simulink model "lss"  (R2022b)
settings: Solver=FixedStepAuto  StartTime=0.0  StopTime=Inf  FixedStep=0.001  RelTol=1e-3  EnableMultiTasking=on
InitFcn:
  | clear mex
model workspace (MAT data in the model file):
  worldsim_instance : object (value not decoded)
values from neighbouring files (symbols this model uses):
  ADAS_Control_Mode = 1    [LSS_parameters.m]    (also in lss_ini_param.sldd = 1.0)
  butter_a = 1.0 -1.9911142922016536 0.99115359586893548    [lss_ini_param.sldd]
  butter_a_lka_out = 1.0 -1.5610180758007179 0.641351538057563    [lss_ini_param.sldd]
  butter_b = 9.825916820482009E-6 1.9651833640964018E-5 9.825916820482009E-6    [lss_ini_param.sldd]
  butter_b_lka_out = 0.020083365564211246 0.040166731128422492 0.020083365564211246    [lss_ini_param.sldd]
  index_variant_approaching_speed = 3.0    [lss_ini_param.sldd]
  initCond = vi_worldsim_load_scenario(worldsim_process,scenario_path,'lss_online')    [launcher.m]
  LDW_Activity_Flag = 1    [LSS_parameters.m]    (also in lss_ini_param.sldd = 1.0)
  LDW_Freq_Hz = Sensor_Freq_worldsim    [LSS_parameters.m]    (also in lss_ini_param.sldd = 50.0)
  LDW_LaneGap_dydt_Warning = 50    [LSS_parameters.m]    (also in lss_ini_param.sldd = 50.0)
  LDW_LaneGap_Warning = [0.5 0.25]    [LSS_parameters.m]    (also in lss_ini_param.sldd = 0.5 0.25)
  LDW_Min_Speed = 60    [LSS_parameters.m]    (also in lss_ini_param.sldd = 60.0)
  LDW_Steer_Vibration_Amplitude = 5    [LSS_parameters.m]    (also in lss_ini_param.sldd = 5.0)
  LDW_Steer_Vibration_Freq = 25    [LSS_parameters.m]    (also in lss_ini_param.sldd = 25.0)
  LKA_Activity_Flag = 1    [LSS_parameters.m]    (also in lss_ini_param.sldd = 1.0)
  LKA_D = [0.2 0.3]    [LSS_parameters.m]    (also in lss_ini_param.sldd = 0.2 0.3)
  LKA_Dyn_Rate_Limiter_Gain = 0.1    [LSS_parameters.m]    (also in lss_ini_param.sldd)
  LKA_Dyn_Rate_Limiter_Power = 10    [LSS_parameters.m]    (also in lss_ini_param.sldd = 10.0)
  LKA_Error_dydt_Off = 1    [LSS_parameters.m]    (also in lss_ini_param.sldd = 1.0)
  LKA_Error_Max = 3    [LSS_parameters.m]    (also in lss_ini_param.sldd = 3.0)
  LKA_Error_Off = 0.5    [LSS_parameters.m]    (also in lss_ini_param.sldd)
  LKA_Freq_Hz = Sensor_Freq_worldsim    [LSS_parameters.m]    (also in lss_ini_param.sldd = 50.0)
  LKA_I = [0.025 0.05]    [LSS_parameters.m]    (also in lss_ini_param.sldd = 0.025 0.05)
  LKA_Lane_Gap_Activate = [0.25 0.125]    [LSS_parameters.m]    (also in lss_ini_param.sldd = -0.05 0.125)
  LKA_Lane_Gap_dydt_Activate = 50    [LSS_parameters.m]    (also in lss_ini_param.sldd = 50.0)
  LKA_Min_Speed = 60    [LSS_parameters.m]    (also in lss_ini_param.mat = 50; lss_ini_param.sldd = 50.0)
  LKA_On_Display_Freq = 5    [LSS_parameters.m]    (also in lss_ini_param.sldd = 5.0)
  LKA_P = [0.1 0.2]    [LSS_parameters.m]    (also in lss_ini_param.sldd = 0.1 0.2)
  LKA_Steer_Rate_Max_radps = 1    [LSS_parameters.m]    (also in lss_ini_param.sldd = 1.0)
  radar_source = 2    [LSS_parameters.m]    (also in lss_ini_param.sldd = 2.0)
  Sensor_Freq_worldsim = 50    [launcher.m]    (also in lss_ini_param.sldd = 50.0)
  simulation_crt = '../VI-CarRealTime_model/SedanCar_WorldSim_Offline_send_svm.xml'    [launcher.m]
  stop_number_collisions = 5    [launcher.m]
  stop_speed = 0.001    [launcher.m]
  stop_time = 20    [launcher.m]
  target_speed = 72    [LSS_parameters.m]    (also in launcher.m = initCond.initialVelocity * 3.6)
  variant_approaching_speed = v_lat    [launcher.m]    (also in lss_ini_param.sldd = 0.2 0.3 0.4 0.5 0.6)
  vehicle_width = 1.86    [LSS_parameters.m]    (also in lss_ini_param.sldd = 2.05)
undefined symbols (not defined in the file or in its folder): Driver_Demands, light_brake_center, light_brake_left, light_brake_right, steer_assist, vicrt_initcallback, vicrt_initmexcallback, vicrt_simulationmanager
libraries: simulink x39, simwbSfunlib x15, viworldsim_lib x5
(part 3 of 6)

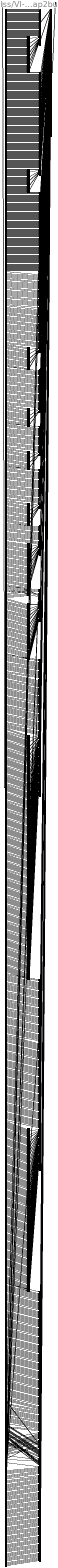
== system lss/VI-CarRealTime/Output_Bus/IOmap2bus ==
  In : Inport
  ABS_Activity : BusCreator  Inputs=4
  Actual_Tread_Speed : BusCreator  Inputs=4
  Aggregate_Force_At_Wheel : BusCreator  Inputs=4
  Alpha : BusCreator  Inputs=4
  Animator_Widget : BusCreator  Inputs=2
  Auxiliary_Roll_Force : BusCreator  Inputs=4
  Auxiliary_Roll_Force_at_element : BusCreator  Inputs=2
  Auxiliary_Roll_deformation_at_element : BusCreator  Inputs=2
  Brake : BusCreator  Inputs=8
  Brake_Moment : BusCreator  Inputs=4
  Caster_Angle : BusCreator  Inputs=2
  Chamber_Pressure : BusCreator  Inputs=4
  Contact_Flag : BusCreator  Inputs=4
  Contact_Patch_Global_X : BusCreator  Inputs=4
  Contact_Patch_Global_X1 : BusCreator  Inputs=4
  Contact_Patch_Global_Y : BusCreator  Inputs=4
  Contact_Patch_Global_Y1 : BusCreator  Inputs=4
  Contact_Patch_Global_Z : BusCreator  Inputs=4
  Contact_Patch_Global_Z1 : BusCreator  Inputs=4
  Contact_Patch_Normal_X : BusCreator  Inputs=4
  Contact_Patch_Normal_Y : BusCreator  Inputs=4
  Contact_Patch_Normal_Z : BusCreator  Inputs=4
  Damper : BusCreator  Inputs=5
  Demux : Demux  Outputs=1377
  Drive_Moment : BusCreator  Inputs=4
  Effective_Closing_Speed : BusCreator  Inputs=4
  Effective_Penetration : BusCreator  Inputs=4
  Effective_Rolling_Radius : BusCreator  Inputs=4
  Equivalent_Tread_Speed : BusCreator  Inputs=4
  Euler_Roll : BusCreator  Inputs=4
  External_Friction_Scale_Factor : BusCreator  Inputs=4
  Force_At_Bumper : BusCreator  Inputs=4
  Force_At_Bumper1 : BusCreator  Inputs=4
  Force_At_Damper : BusCreator  Inputs=4
  Force_At_Inerter : BusCreator  Inputs=4
  Force_At_Spring : BusCreator  Inputs=4
  Force_At_Wheel{,1..4} (5 alike) : BusCreator  Inputs=4
  Force_Aux_At_Wheel : BusCreator  Inputs=4
  Global_Omega_X : BusCreator  Inputs=4
  Global_Omega_Y : BusCreator  Inputs=4
  Global_Omega_Z : BusCreator  Inputs=4
  Global_Vx : BusCreator  Inputs=4
  Global_Vy : BusCreator  Inputs=4
  Global_Vz : BusCreator  Inputs=4
  Global_X : BusCreator  Inputs=4
  Global_Y : BusCreator  Inputs=4
  Global_Z : BusCreator  Inputs=4
  Ground_Surface_Contact_Patch_Vx : BusCreator  Inputs=4
  Ground_Surface_Contact_Patch_Vy : BusCreator  Inputs=4
  Ground_Surface_Force_X : BusCreator  Inputs=4
  Ground_Surface_Force_Y : BusCreator  Inputs=4
  Ground_Surface_Force_Z : BusCreator  Inputs=4
  Ground_Surface_Gyroscopic_Moment : BusCreator  Inputs=4
  Ground_Surface_Kappa_Fy : BusCreator  Inputs=4
  Ground_Surface_Moment_X : BusCreator  Inputs=4
  Ground_Surface_Moment_Y : BusCreator  Inputs=4
  Ground_Surface_Moment_Z : BusCreator  Inputs=4
  Ground_Surface_Peak_Friction_X : BusCreator  Inputs=4
  Ground_Surface_Peak_Friction_Y : BusCreator  Inputs=4
  Ground_Surface_Residual_Torque : BusCreator  Inputs=4
  Ground_Surface_Wheel_Center_Vx : BusCreator  Inputs=4
  Gyro : BusCreator  Inputs=10
  Hook_rear : BusCreator  Inputs=18
  Hub_Carrier_Force_Global_X : BusCreator  Inputs=4
  Hub_Carrier_Force_Global_Y : BusCreator  Inputs=4
  Hub_Carrier_Force_Global_Z : BusCreator  Inputs=4
  Hub_Carrier_Force_Local_X : BusCreator  Inputs=4
  Hub_Carrier_Force_Local_Y : BusCreator  Inputs=4
  Hub_Carrier_Force_Local_Z : BusCreator  Inputs=4
  Hub_Carrier_Moment_Global_X : BusCreator  Inputs=4
  Hub_Carrier_Moment_Global_Y : BusCreator  Inputs=4
  Hub_Carrier_Moment_Global_Z : BusCreator  Inputs=4
  Hub_Carrier_Moment_Local_X : BusCreator  Inputs=4
  Hub_Carrier_Moment_Local_Y : BusCreator  Inputs=4
  Hub_Carrier_Moment_Local_Z : BusCreator  Inputs=4
  Hub_Carrier_Omega_X : BusCreator  Inputs=4
  Hub_Carrier_Omega_Y : BusCreator  Inputs=4
  Hub_Carrier_Omega_Z : BusCreator  Inputs=4
  Hub_Carrier_Vx : BusCreator  Inputs=4
  Hub_Carrier_Vy : BusCreator  Inputs=4
  Hub_Carrier_Vz : BusCreator  Inputs=4
  Inclination : BusCreator  Inputs=4
  Inerter : BusCreator  Inputs=5
  Inst_Stiff_Deflection : BusCreator  Inputs=4
  Inst_Stiff_Force : BusCreator  Inputs=4
  Jounce{,1..5} (6 alike) : BusCreator  Inputs=4
  Jounce_Acceleration{,1..3} (4 alike) : BusCreator  Inputs=4
  Jounce_Bumper : BusCreator  Inputs=4
  Jounce_Rate{,1..5} (6 alike) : BusCreator  Inputs=4
  Kingpin_Moment : BusCreator  Inputs=1
  Kingpin_Moment1 : BusCreator  Inputs=2
  Lateral_Relaxation_Length : BusCreator  Inputs=4
  Lateral_Slip_With_Lag : BusCreator  Inputs=4
  Lateral_Slip_Without_Lag : BusCreator  Inputs=4
  Loaded_Radius : BusCreator  Inputs=4
  Locked_Damper_Moment : BusCreator  Inputs=4
  Locked_Moment : BusCreator  Inputs=4
  Locked_Spring_Moment : BusCreator  Inputs=4
  Locked_Switch : BusCreator  Inputs=4
  Lockup_Rotation : BusCreator  Inputs=4
  Longitudinal_Relaxation_Length : BusCreator  Inputs=4
  Longitudinal_Slip_With_Lag : BusCreator  Inputs=4
  Longitudinal_Slip_Without_Lag : BusCreator  Inputs=4
  Moment_Arm_Of_Fx : BusCreator  Inputs=4
  Motor : BusCreator  Inputs=5
  Off_Road_Flag : BusCreator  Inputs=4
  Omega : BusCreator  Inputs=4
  OutputBus : BusCreator  Inputs=113
  PID_CW_At_Spring : BusCreator  Inputs=4
  PID_PH_At_Spring : BusCreator  Inputs=4
  PID_RH_At_Spring : BusCreator  Inputs=4
  Phi : BusCreator  Inputs=4
  Pitch : BusCreator  Inputs=4
  Pneumatic_Trail : BusCreator  Inputs=4
  Pressure : BusCreator  Inputs=4
  Psi : BusCreator  Inputs=4
  Rebound_Bumper : BusCreator  Inputs=4
  Road : BusCreator  Inputs=5
  Road_Material : BusCreator  Inputs=4
  Road_friction : BusCreator  Inputs=4
  Roll : BusCreator  Inputs=2
  Roll_Center_Height : BusCreator  Inputs=2
  Roll_Center_Lateral_Displacement : BusCreator  Inputs=2
  Rotation : BusCreator  Inputs=4
  Sensor : BusCreator  Inputs=16
  Side_View_Angle : BusCreator  Inputs=4
  Spindle_Steer : BusCreator  Inputs=4
  Spring : BusCreator  Inputs=10
  Steering_Column : BusCreator  Inputs=32
  Steering_Instant_Axis_Rotation : BusCreator  Inputs=2
  Steering_Rack_Pinion : BusCreator  Inputs=11
  Steering_System : BusCreator  Inputs=13
  Steering_Torsion_Bar : BusCreator  Inputs=5
  Suspension : BusCreator  Inputs=16
  System : BusCreator  Inputs=18
  System_Mass_Center : BusCreator  Inputs=13
  Temperature_{1..4} (4 alike) : BusCreator  Inputs=4
  Theta : BusCreator  Inputs=4
  TieRod_Force_Left : BusCreator  Inputs=3
  TieRod_Force_Right : BusCreator  Inputs=3
  Tire : BusCreator  Inputs=54
  Tire_front_left : BusCreator  Inputs=6
  Tire_front_right : BusCreator  Inputs=6
  Tire_rear_left : BusCreator  Inputs=6
  Tire_rear_right : BusCreator  Inputs=6
  User_Input_Contact_Patch_Global_Z_Perturbation : BusCreator  Inputs=4
  Vehicle : BusCreator  Inputs=46
  Vehicle_States : BusCreator  Inputs=20
  Wear : BusCreator  Inputs=4
  Wheel : BusCreator  Inputs=37
  Yaw : BusCreator  Inputs=4
  aero_forces : BusCreator  Inputs=24
  base_acceleration : BusCreator  Inputs=4
  base_deformation : BusCreator  Inputs=4
  base_velocity : BusCreator  Inputs=4
  bul_jounce_stop_data : BusCreator  Inputs=6
  bul_rebound_stop_data : BusCreator  Inputs=6
  bur_jounce_stop_data : BusCreator  Inputs=6
  bur_rebound_stop_data : BusCreator  Inputs=6
  bus_dmp_jounce_stop_data : BusCreator  Inputs=6
  bus_ins_jounce_stop_data : BusCreator  Inputs=6
  bus_roll_dmp_jounce_stop_data : BusCreator  Inputs=6
  bus_spr_jounce_stop_data : BusCreator  Inputs=6
  chassis_accelerations : BusCreator  Inputs=6
  chassis_displacements : BusCreator  Inputs=9
  chassis_velocities : BusCreator  Inputs=6
  clutch : BusCreator  Inputs=8
  condition_sensors : BusCreator  Inputs=1
  cp_force_lateralFL : BusCreator  Inputs=3
  cp_force_lateralFR : BusCreator  Inputs=3
  cp_force_lateralRL : BusCreator  Inputs=3
  cp_force_lateralRR : BusCreator  Inputs=3
  cp_force_longitudinalFL : BusCreator  Inputs=3
  cp_force_longitudinalFR : BusCreator  Inputs=3
  cp_force_longitudinalRL : BusCreator  Inputs=3
  cp_force_longitudinalRR : BusCreator  Inputs=3
  cp_force_normalFL : BusCreator  Inputs=3
  cp_force_normalFR : BusCreator  Inputs=3
  cp_force_normalRL : BusCreator  Inputs=3
  cp_force_normalRR : BusCreator  Inputs=3
  cross_weight : BusCreator  Inputs=4
  dal_ride_damper_data : BusCreator  Inputs=4
  dar_ride_damper_data : BusCreator  Inputs=4
  das_ride_damper_data : BusCreator  Inputs=6
  das_roll_damper_data : BusCreator  Inputs=8
  das_third_damper_data : BusCreator  Inputs=6
  differential_central : BusCreator  Inputs=7
  differential_front : BusCreator  Inputs=7
  differential_rear : BusCreator  Inputs=7
  differential_speeds : BusCreator  Inputs=9
  differential_torques : BusCreator  Inputs=9
  driver_demands : BusCreator  Inputs=9
  driving_machine_monitor : BusCreator  Inputs=15
  engine : BusCreator  Inputs=11
  fuel_consumption : BusCreator  Inputs=5
  ges_chassis_XFORM : BusCreator  Inputs=6
  ges_hub_XFORMFL : BusCreator  Inputs=6
  ges_hub_XFORMFR : BusCreator  Inputs=6
  ges_hub_XFORMRL : BusCreator  Inputs=6
  ges_hub_XFORMRR : BusCreator  Inputs=6
  hub2cp_XFORMFL : BusCreator  Inputs=3
  hub2cp_XFORMFR : BusCreator  Inputs=3
  hub2cp_XFORMRL : BusCreator  Inputs=3
  hub2cp_XFORMRR : BusCreator  Inputs=3
  hub_center_accx : BusCreator  Inputs=4
  hub_center_accy : BusCreator  Inputs=4
  hub_center_accz : BusCreator  Inputs=4
  inl_ride_inerter_data : BusCreator  Inputs=6
  inr_ride_inerter_data : BusCreator  Inputs=6
  ins_inerter_data : BusCreator  Inputs=10
  jfs_torsional_stiffness_data : BusCreator  Inputs=12
  nsl_ride_spring_data : BusCreator  Inputs=6
  nsr_ride_spring_data : BusCreator  Inputs=6
  nss_ride_spring_data : BusCreator  Inputs=10
  path_sensor : BusCreator  Inputs=6
  res_dmp_rebound_stop_data : BusCreator  Inputs=6
  res_ins_rebound_stop_data : BusCreator  Inputs=6
  res_roll_dmp_rebound_stop_data : BusCreator  Inputs=6
  res_spr_rebound_stop_data : BusCreator  Inputs=6
  rhl_front_setup_sensor_data : BusCreator  Inputs=1
  rhl_rear_setup_sensor_data : BusCreator  Inputs=1
  rhr_front_setup_sensor_data : BusCreator  Inputs=1
  rhr_rear_setup_sensor_data : BusCreator  Inputs=1
  rhs_front_setup_sensor_data : BusCreator  Inputs=1
  rhs_rear_setup_sensor_data : BusCreator  Inputs=1
  til_wheel_tire_forces : BusCreator  Inputs=18
  til_wheel_tire_kinematics : BusCreator  Inputs=9
  til_wheel_tire_rolling_states : BusCreator  Inputs=9
  tir_wheel_tire_forces : BusCreator  Inputs=18
  tir_wheel_tire_kinematics : BusCreator  Inputs=9
  tir_wheel_tire_rolling_states : BusCreator  Inputs=9
  torque_converter : BusCreator  Inputs=9
  transmission : BusCreator  Inputs=11
  ues_third_spring_data : BusCreator  Inputs=6
  upright_accelerometer : BusCreator  Inputs=4
  wheel_angles : BusCreator  Inputs=24
  wheel_center_dispx : BusCreator  Inputs=4
  wheel_center_dispy : BusCreator  Inputs=4
  wheel_center_dispz : BusCreator  Inputs=4
  whl_front_wheel_XFORM : BusCreator  Inputs=9
  whl_rear_wheel_XFORM : BusCreator  Inputs=9
  whl_twin_rear_wheel_XFORM : BusCreator  Inputs=9
  whr_front_wheel_XFORM : BusCreator  Inputs=9
  whr_rear_wheel_XFORM : BusCreator  Inputs=9
  whr_twin_rear_wheel_XFORM : BusCreator  Inputs=9
  Out : Outport
  wires:
  In/1 -> Demux/1
  OutputBus/1 -> Out/1  "OutputBus"
  aero_forces/1 -> OutputBus/1  "aero_forces"
  Demux/1 -> aero_forces/1  "aero_balance"
  Demux/2 -> aero_forces/2  "center_downforce"
  Demux/3 -> aero_forces/3  "center_sideforce"
  Demux/4 -> aero_forces/4  "drag_arm"
  Demux/5 -> aero_forces/5  "drag_force"
  Demux/6 -> aero_forces/6  "drag_force_front"
  Demux/7 -> aero_forces/7  "drag_force_rear"
  Demux/8 -> aero_forces/8  "drag_torque"
  Demux/9 -> aero_forces/9  "front_downforce"
  Demux/10 -> aero_forces/10  "front_sideforce"
  Demux/11 -> aero_forces/11  "height_auxiliary"
  Demux/12 -> aero_forces/12  "height_front"
  Demux/13 -> aero_forces/13  "height_rear"
  Demux/14 -> aero_forces/14  "lateral_velocity"
  Demux/15 -> aero_forces/15  "longitudinal_velocity"
  Demux/16 -> aero_forces/16  "pitch"
  Demux/17 -> aero_forces/17  "rear_downforce"
  Demux/18 -> aero_forces/18  "rear_sideforce"
  Demux/19 -> aero_forces/19  "roll"
  Demux/20 -> aero_forces/20  "roll_torque"
  Demux/21 -> aero_forces/21  "side_slip"
  Demux/22 -> aero_forces/22  "steer"
  Demux/23 -> aero_forces/23  "vertical_velocity"
  Demux/24 -> aero_forces/24  "yaw_torque"
  Brake/1 -> OutputBus/2  "Brake"
  ABS_Activity/1 -> Brake/1  "ABS_Activity"
  Demux/25 -> ABS_Activity/1  "L1"
  Demux/26 -> ABS_Activity/2  "L2"
  Demux/27 -> ABS_Activity/3  "R1"
  Demux/28 -> ABS_Activity/4  "R2"
  Brake_Moment/1 -> Brake/2  "Brake_Moment"
  Demux/29 -> Brake_Moment/1  "L1"
  Demux/30 -> Brake_Moment/2  "L2"
  Demux/31 -> Brake_Moment/3  "R1"
  Demux/32 -> Brake_Moment/4  "R2"
  Chamber_Pressure/1 -> Brake/3  "Chamber_Pressure"
  Demux/33 -> Chamber_Pressure/1  "L1"
  Demux/34 -> Chamber_Pressure/2  "L2"
  Demux/35 -> Chamber_Pressure/3  "R1"
  Demux/36 -> Chamber_Pressure/4  "R2"
  Locked_Damper_Moment/1 -> Brake/4  "Locked_Damper_Moment"
  Demux/37 -> Locked_Damper_Moment/1  "L1"
  Demux/38 -> Locked_Damper_Moment/2  "L2"
  Demux/39 -> Locked_Damper_Moment/3  "R1"
  Demux/40 -> Locked_Damper_Moment/4  "R2"
  Locked_Moment/1 -> Brake/5  "Locked_Moment"
  Demux/41 -> Locked_Moment/1  "L1"
  Demux/42 -> Locked_Moment/2  "L2"
  Demux/43 -> Locked_Moment/3  "R1"
  Demux/44 -> Locked_Moment/4  "R2"
  Locked_Spring_Moment/1 -> Brake/6  "Locked_Spring_Moment"
  Demux/45 -> Locked_Spring_Moment/1  "L1"
  Demux/46 -> Locked_Spring_Moment/2  "L2"
  Demux/47 -> Locked_Spring_Moment/3  "R1"
  Demux/48 -> Locked_Spring_Moment/4  "R2"
  Locked_Switch/1 -> Brake/7  "Locked_Switch"
  Demux/49 -> Locked_Switch/1  "L1"
  Demux/50 -> Locked_Switch/2  "L2"
  Demux/51 -> Locked_Switch/3  "R1"
  Demux/52 -> Locked_Switch/4  "R2"
  Lockup_Rotation/1 -> Brake/8  "Lockup_Rotation"
  Demux/53 -> Lockup_Rotation/1  "L1"
  Demux/54 -> Lockup_Rotation/2  "L2"
  Demux/55 -> Lockup_Rotation/3  "R1"
  Demux/56 -> Lockup_Rotation/4  "R2"
  bul_jounce_stop_data/1 -> OutputBus/3  "bul_jounce_stop_data"
  Demux/57 -> bul_jounce_stop_data/1  "force_front"
  Demux/58 -> bul_jounce_stop_data/2  "force_rear"
  Demux/59 -> bul_jounce_stop_data/3  "jounce_front"
  Demux/60 -> bul_jounce_stop_data/4  "jounce_rear"
  Demux/61 -> bul_jounce_stop_data/5  "velocity_front"
  Demux/62 -> bul_jounce_stop_data/6  "velocity_rear"
  bul_rebound_stop_data/1 -> OutputBus/4  "bul_rebound_stop_data"
  Demux/63 -> bul_rebound_stop_data/1  "force_front"
  Demux/64 -> bul_rebound_stop_data/2  "force_rear"
  Demux/65 -> bul_rebound_stop_data/3  "jounce_front"
  Demux/66 -> bul_rebound_stop_data/4  "jounce_rear"
  Demux/67 -> bul_rebound_stop_data/5  "velocity_front"
  Demux/68 -> bul_rebound_stop_data/6  "velocity_rear"
  bur_jounce_stop_data/1 -> OutputBus/5  "bur_jounce_stop_data"
  Demux/69 -> bur_jounce_stop_data/1  "force_front"
  Demux/70 -> bur_jounce_stop_data/2  "force_rear"
  Demux/71 -> bur_jounce_stop_data/3  "jounce_front"
  Demux/72 -> bur_jounce_stop_data/4  "jounce_rear"
  Demux/73 -> bur_jounce_stop_data/5  "velocity_front"
  Demux/74 -> bur_jounce_stop_data/6  "velocity_rear"
  bur_rebound_stop_data/1 -> OutputBus/6  "bur_rebound_stop_data"
  Demux/75 -> bur_rebound_stop_data/1  "force_front"
  Demux/76 -> bur_rebound_stop_data/2  "force_rear"
  Demux/77 -> bur_rebound_stop_data/3  "jounce_front"
  Demux/78 -> bur_rebound_stop_data/4  "jounce_rear"
  Demux/79 -> bur_rebound_stop_data/5  "velocity_front"
  Demux/80 -> bur_rebound_stop_data/6  "velocity_rear"
  bus_dmp_jounce_stop_data/1 -> OutputBus/7  "bus_dmp_jounce_stop_data"
  Demux/81 -> bus_dmp_jounce_stop_data/1  "displacement_front"
  Demux/82 -> bus_dmp_jounce_stop_data/2  "displacement_rear"
  Demux/83 -> bus_dmp_jounce_stop_data/3  "force_front"
  Demux/84 -> bus_dmp_jounce_stop_data/4  "force_rear"
  Demux/85 -> bus_dmp_jounce_stop_data/5  "velocity_front"
  Demux/86 -> bus_dmp_jounce_stop_data/6  "velocity_rear"
  bus_ins_jounce_stop_data/1 -> OutputBus/8  "bus_ins_jounce_stop_data"
  Demux/87 -> bus_ins_jounce_stop_data/1  "displacement_front"
  Demux/88 -> bus_ins_jounce_stop_data/2  "displacement_rear"
  Demux/89 -> bus_ins_jounce_stop_data/3  "force_front"
  Demux/90 -> bus_ins_jounce_stop_data/4  "force_rear"
  Demux/91 -> bus_ins_jounce_stop_data/5  "velocity_front"
  Demux/92 -> bus_ins_jounce_stop_data/6  "velocity_rear"
  bus_roll_dmp_jounce_stop_data/1 -> OutputBus/9  "bus_roll_dmp_jounce_stop_data"
  Demux/93 -> bus_roll_dmp_jounce_stop_data/1  "displacement_front"
  Demux/94 -> bus_roll_dmp_jounce_stop_data/2  "displacement_rear"
  Demux/95 -> bus_roll_dmp_jounce_stop_data/3  "force_front"
  Demux/96 -> bus_roll_dmp_jounce_stop_data/4  "force_rear"
  Demux/97 -> bus_roll_dmp_jounce_stop_data/5  "velocity_front"
  Demux/98 -> bus_roll_dmp_jounce_stop_data/6  "velocity_rear"
  bus_spr_jounce_stop_data/1 -> OutputBus/10  "bus_spr_jounce_stop_data"
  Demux/99 -> bus_spr_jounce_stop_data/1  "displacement_front"
  Demux/100 -> bus_spr_jounce_stop_data/2  "displacement_rear"
  Demux/101 -> bus_spr_jounce_stop_data/3  "force_front"
  Demux/102 -> bus_spr_jounce_stop_data/4  "force_rear"
  Demux/103 -> bus_spr_jounce_stop_data/5  "velocity_front"
  Demux/104 -> bus_spr_jounce_stop_data/6  "velocity_rear"
  chassis_accelerations/1 -> OutputBus/11  "chassis_accelerations"
  Demux/105 -> chassis_accelerations/1  "lateral"
  Demux/106 -> chassis_accelerations/2  "longitudinal"
  Demux/107 -> chassis_accelerations/3  "pitch"
  Demux/108 -> chassis_accelerations/4  "roll"
  Demux/109 -> chassis_accelerations/5  "vertical"
  Demux/110 -> chassis_accelerations/6  "yaw"
  chassis_displacements/1 -> OutputBus/12  "chassis_displacements"
  Demux/111 -> chassis_displacements/1  "lateral"
  Demux/112 -> chassis_displacements/2  "longitudinal"
  Demux/113 -> chassis_displacements/3  "pitch"
  Demux/114 -> chassis_displacements/4  "pitch_wrt_road"
  Demux/115 -> chassis_displacements/5  "roll"
  Demux/116 -> chassis_displacements/6  "roll_wrt_road"
  Demux/117 -> chassis_displacements/7  "vertical"
  Demux/118 -> chassis_displacements/8  "vertical_wrt_road"
  Demux/119 -> chassis_displacements/9  "yaw"
  chassis_velocities/1 -> OutputBus/13  "chassis_velocities"
  Demux/120 -> chassis_velocities/1  "lateral"
  Demux/121 -> chassis_velocities/2  "longitudinal"
  Demux/122 -> chassis_velocities/3  "pitch"
  Demux/123 -> chassis_velocities/4  "roll"
  Demux/124 -> chassis_velocities/5  "vertical"
  Demux/125 -> chassis_velocities/6  "yaw"
  clutch/1 -> OutputBus/14  "clutch"
  Demux/126 -> clutch/1  "clutch_rpm"
  Demux/127 -> clutch/2  "effective_clutch"
  Demux/128 -> clutch/3  "gearbox_inputshaft_alpha"
  Demux/129 -> clutch/4  "gearbox_inputshaft_angle"
  Demux/130 -> clutch/5  "gearbox_inputshaft_omega"
  Demux/131 -> clutch/6  "inputplate_torque"
  Demux/132 -> clutch/7  "slip_angle"
  Demux/133 -> clutch/8  "torque"
  condition_sensors/1 -> OutputBus/15  "condition_sensors"
  Demux/134 -> condition_sensors/1  "side_slip_angle"
  cross_weight/1 -> OutputBus/16  "cross_weight"
  Demux/135 -> cross_weight/1  "crossL1R2_ratio"
  Demux/136 -> cross_weight/2  "crossR1L2_ratio"
  Demux/137 -> cross_weight/3  "nose_ratio"
  Demux/138 -> cross_weight/4  "side_right_ratio"
  dal_ride_damper_data/1 -> OutputBus/17  "dal_ride_damper_data"
  Demux/139 -> dal_ride_damper_data/1  "force_front"
  Demux/140 -> dal_ride_damper_data/2  "force_rear"
  Demux/141 -> dal_ride_damper_data/3  "velocity_front"
  Demux/142 -> dal_ride_damper_data/4  "velocity_rear"
  Damper/1 -> OutputBus/18  "Damper"
  Force_At_Damper/1 -> Damper/1  "Force_At_Damper"
  Demux/143 -> Force_At_Damper/1  "L1"
  Demux/144 -> Force_At_Damper/2  "L2"
  Demux/145 -> Force_At_Damper/3  "R1"
  Demux/146 -> Force_At_Damper/4  "R2"
  Force_At_Wheel/1 -> Damper/2  "Force_At_Wheel"
  Demux/147 -> Force_At_Wheel/1  "L1"
  Demux/148 -> Force_At_Wheel/2  "L2"
  Demux/149 -> Force_At_Wheel/3  "R1"
  Demux/150 -> Force_At_Wheel/4  "R2"
  Jounce/1 -> Damper/3  "Jounce"
  Demux/151 -> Jounce/1  "L1"
  Demux/152 -> Jounce/2  "L2"
  Demux/153 -> Jounce/3  "R1"
  Demux/154 -> Jounce/4  "R2"
  Jounce_Acceleration/1 -> Damper/4  "Jounce_Acceleration"
  Demux/155 -> Jounce_Acceleration/1  "L1"
  Demux/156 -> Jounce_Acceleration/2  "L2"
  Demux/157 -> Jounce_Acceleration/3  "R1"
  Demux/158 -> Jounce_Acceleration/4  "R2"
  Jounce_Rate/1 -> Damper/5  "Jounce_Rate"
  Demux/159 -> Jounce_Rate/1  "L1"
  Demux/160 -> Jounce_Rate/2  "L2"
  Demux/161 -> Jounce_Rate/3  "R1"
  Demux/162 -> Jounce_Rate/4  "R2"
  dar_ride_damper_data/1 -> OutputBus/19  "dar_ride_damper_data"
  Demux/163 -> dar_ride_damper_data/1  "force_front"
  Demux/164 -> dar_ride_damper_data/2  "force_rear"
  Demux/165 -> dar_ride_damper_data/3  "velocity_front"
  Demux/166 -> dar_ride_damper_data/4  "velocity_rear"
  das_ride_damper_data/1 -> OutputBus/20  "das_ride_damper_data"
  Demux/167 -> das_ride_damper_data/1  "displacement_front"
  Demux/168 -> das_ride_damper_data/2  "displacement_rear"
  Demux/169 -> das_ride_damper_data/3  "force_front"
  Demux/170 -> das_ride_damper_data/4  "force_rear"
  Demux/171 -> das_ride_damper_data/5  "velocity_front"
  Demux/172 -> das_ride_damper_data/6  "velocity_rear"
  das_roll_damper_data/1 -> OutputBus/21  "das_roll_damper_data"
  Demux/173 -> das_roll_damper_data/1  "displacement_front"
  Demux/174 -> das_roll_damper_data/2  "displacement_rear"
  Demux/175 -> das_roll_damper_data/3  "force_at_wheel_front"
  Demux/176 -> das_roll_damper_data/4  "force_at_wheel_rear"
  Demux/177 -> das_roll_damper_data/5  "force_front"
  Demux/178 -> das_roll_damper_data/6  "force_rear"
  Demux/179 -> das_roll_damper_data/7  "velocity_front"
  Demux/180 -> das_roll_damper_data/8  "velocity_rear"
  das_third_damper_data/1 -> OutputBus/22  "das_third_damper_data"
  Demux/181 -> das_third_damper_data/1  "displacement_front"
  Demux/182 -> das_third_damper_data/2  "displacement_rear"
  Demux/183 -> das_third_damper_data/3  "force_front"
  Demux/184 -> das_third_damper_data/4  "force_rear"
  Demux/185 -> das_third_damper_data/5  "velocity_front"
  Demux/186 -> das_third_damper_data/6  "velocity_rear"
  differential_central/1 -> OutputBus/23  "differential_central"
  Demux/187 -> differential_central/1  "diff_front_inputshaft_alpha"
  Demux/188 -> differential_central/2  "diff_front_inputshaft_angle"
  Demux/189 -> differential_central/3  "diff_front_inputshaft_omega"
  Demux/190 -> differential_central/4  "diff_rear_inputshaft_alpha"
  Demux/191 -> differential_central/5  "diff_rear_inputshaft_angle"
  Demux/192 -> differential_central/6  "diff_rear_inputshaft_omega"
  Demux/193 -> differential_central/7  "gearbox_outputshaft_torque"
  differential_front/1 -> OutputBus/24  "differential_front"
  Demux/194 -> differential_front/1  "diff_central_front_outputshaft_torque"
  Demux/195 -> differential_front/2  "wheel_front_left_alpha"
  Demux/196 -> differential_front/3  "wheel_front_left_angle"
  Demux/197 -> differential_front/4  "wheel_front_left_omega"
  Demux/198 -> differential_front/5  "wheel_front_right_alpha"
  Demux/199 -> differential_front/6  "wheel_front_right_angle"
  Demux/200 -> differential_front/7  "wheel_front_right_omega"
  differential_rear/1 -> OutputBus/25  "differential_rear"
  Demux/201 -> differential_rear/1  "diff_central_rear_outputshaft_torque"
  Demux/202 -> differential_rear/2  "wheel_rear_left_alpha"
  Demux/203 -> differential_rear/3  "wheel_rear_left_angle"
  Demux/204 -> differential_rear/4  "wheel_rear_left_omega"
  Demux/205 -> differential_rear/5  "wheel_rear_right_alpha"
  Demux/206 -> differential_rear/6  "wheel_rear_right_angle"
  Demux/207 -> differential_rear/7  "wheel_rear_right_omega"
  differential_speeds/1 -> OutputBus/26  "differential_speeds"
  Demux/208 -> differential_speeds/1  "halfshaft_omega_central_front"
  Demux/209 -> differential_speeds/2  "halfshaft_omega_central_rear"
  Demux/210 -> differential_speeds/3  "halfshaft_omega_delta_central"
  Demux/211 -> differential_speeds/4  "halfshaft_omega_delta_front"
  Demux/212 -> differential_speeds/5  "halfshaft_omega_delta_rear"
  Demux/213 -> differential_speeds/6  "halfshaft_omega_left_front"
  Demux/214 -> differential_speeds/7  "halfshaft_omega_left_rear"
  Demux/215 -> differential_speeds/8  "halfshaft_omega_right_front"
  Demux/216 -> differential_speeds/9  "halfshaft_omega_right_rear"
  differential_torques/1 -> OutputBus/27  "differential_torques"
  Demux/217 -> differential_torques/1  "differential_torque_central"
  Demux/218 -> differential_torques/2  "differential_torque_front"
  Demux/219 -> differential_torques/3  "differential_torque_rear"
  Demux/220 -> differential_torques/4  "output_torque_central_front"
  Demux/221 -> differential_torques/5  "output_torque_central_rear"
  Demux/222 -> differential_torques/6  "output_torque_left_front"
  Demux/223 -> differential_torques/7  "output_torque_left_rear"
  Demux/224 -> differential_torques/8  "output_torque_right_front"
  Demux/225 -> differential_torques/9  "output_torque_right_rear"
  driver_demands/1 -> OutputBus/28  "driver_demands"
  Demux/226 -> driver_demands/1  "brake"
  Demux/227 -> driver_demands/2  "brake_pressure"
  Demux/228 -> driver_demands/3  "clutch"
  Demux/229 -> driver_demands/4  "gear"
  Demux/230 -> driver_demands/5  "steering"
  Demux/231 -> driver_demands/6  "steering_velocity"
  Demux/232 -> driver_demands/7  "throttle"
  Demux/1233 -> driver_demands/8  "steering_acceleration"
  Demux/1281 -> driver_demands/9  "driver_steering_angle"
  driving_machine_monitor/1 -> OutputBus/29  "driving_machine_monitor"
  Demux/233 -> driving_machine_monitor/1  "driver_brake"
  Demux/234 -> driving_machine_monitor/2  "driver_clutch"
  Demux/235 -> driving_machine_monitor/3  "driver_gear"
  Demux/236 -> driving_machine_monitor/4  "driver_steering"
  Demux/237 -> driving_machine_monitor/5  "driver_throttle"
  Demux/238 -> driving_machine_monitor/6  "maneuver_ID"
  Demux/239 -> driving_machine_monitor/7  "path_curvature"
  Demux/240 -> driving_machine_monitor/8  "path_distance"
  Demux/241 -> driving_machine_monitor/9  "path_s"
  Demux/242 -> driving_machine_monitor/10  "path_x"
  Demux/243 -> driving_machine_monitor/11  "path_y"
  Demux/244 -> driving_machine_monitor/12  "path_z"
  Demux/245 -> driving_machine_monitor/13  "target_ax"
  Demux/246 -> driving_machine_monitor/14  "target_engine_torque"
  Demux/247 -> driving_machine_monitor/15  "target_vx"
  engine/1 -> OutputBus/30  "engine"
  Demux/248 -> engine/1  "clutch_inputplate_alpha"
  Demux/249 -> engine/2  "clutch_inputplate_angle"
  Demux/250 -> engine/3  "clutch_inputplate_omega"
  Demux/251 -> engine/4  "effective_throttle"
  Demux/252 -> engine/5  "engine_rpm"
  Demux/253 -> engine/6  "Max_Engine_torque"
  Demux/254 -> engine/7  "Min_engine_torque"
  Demux/255 -> engine/8  "Power_HP"
  Demux/256 -> engine/9  "Power_KW"
  Demux/257 -> engine/10  "TCS_activity"
  Demux/258 -> engine/11  "torque"
  fuel_consumption/1 -> OutputBus/31  "fuel_consumption"
  Demux/259 -> fuel_consumption/1  "BSFC"
  Demux/260 -> fuel_consumption/2  "instantaneous"
  Demux/261 -> fuel_consumption/3  "instantaneous_Liter_100km"
  Demux/262 -> fuel_consumption/4  "overall"
  Demux/1291 -> fuel_consumption/5  "fuel_mass"
  ges_chassis_XFORM/1 -> OutputBus/32  "ges_chassis_XFORM"
  Demux/263 -> ges_chassis_XFORM/1  "Phi"
  Demux/264 -> ges_chassis_XFORM/2  "Psi"
  Demux/265 -> ges_chassis_XFORM/3  "Theta"
  Demux/266 -> ges_chassis_XFORM/4  "X"
  Demux/267 -> ges_chassis_XFORM/5  "Y"
  Demux/268 -> ges_chassis_XFORM/6  "Z"
  Gyro/1 -> OutputBus/33  "Gyro"
  Demux/269 -> Gyro/1  "Driver_X"
  Demux/270 -> Gyro/2  "Driver_Z"
  Demux/271 -> Gyro/3  "gyro_ACCX"
  Demux/272 -> Gyro/4  "gyro_ACCY"
  Demux/273 -> Gyro/5  "gyro_VX"
  Demux/274 -> Gyro/6  "gyro_X"
  Demux/275 -> Gyro/7  "gyro_Y"
  Demux/276 -> Gyro/8  "sensor_1_Z"
  Demux/277 -> Gyro/9  "sensor_2_Z"
  Demux/278 -> Gyro/10  "sensor_3_Z"
  Hook_rear/1 -> OutputBus/34  "Hook_rear"
  Demux/279 -> Hook_rear/1  "Global_force_X"
  Demux/280 -> Hook_rear/2  "Global_force_Y"
  Demux/281 -> Hook_rear/3  "Global_force_Z"
  Demux/282 -> Hook_rear/4  "Global_Moment_X"
  Demux/283 -> Hook_rear/5  "Global_Moment_Y"
  Demux/284 -> Hook_rear/6  "Global_Moment_Z"
  Demux/285 -> Hook_rear/7  "Hook_Phi"
  Demux/286 -> Hook_rear/8  "Hook_Psi"
  Demux/287 -> Hook_rear/9  "Hook_Theta"
  Demux/288 -> Hook_rear/10  "Hook_X"
  Demux/289 -> Hook_rear/11  "Hook_Y"
  Demux/290 -> Hook_rear/12  "Hook_Z"
  Demux/291 -> Hook_rear/13  "Local_force_X"
  Demux/292 -> Hook_rear/14  "Local_force_Y"
  Demux/293 -> Hook_rear/15  "Local_force_Z"
  Demux/294 -> Hook_rear/16  "Local_Moment_X"
  Demux/295 -> Hook_rear/17  "Local_Moment_Y"
  Demux/296 -> Hook_rear/18  "Local_Moment_Z"
  Inerter/1 -> OutputBus/35  "Inerter"
  Force_At_Inerter/1 -> Inerter/1  "Force_At_Inerter"
  Demux/297 -> Force_At_Inerter/1  "L1"
  Demux/298 -> Force_At_Inerter/2  "L2"
  Demux/299 -> Force_At_Inerter/3  "R1"
  Demux/300 -> Force_At_Inerter/4  "R2"
  Force_At_Wheel1/1 -> Inerter/2  "Force_At_Wheel"
  Demux/301 -> Force_At_Wheel1/1  "L1"
  Demux/302 -> Force_At_Wheel1/2  "L2"
  Demux/303 -> Force_At_Wheel1/3  "R1"
  Demux/304 -> Force_At_Wheel1/4  "R2"
  Jounce1/1 -> Inerter/3  "Jounce"
  Demux/305 -> Jounce1/1  "L1"
  Demux/306 -> Jounce1/2  "L2"
  Demux/307 -> Jounce1/3  "R1"
  Demux/308 -> Jounce1/4  "R2"
  Jounce_Acceleration1/1 -> Inerter/4  "Jounce_Acceleration"
  Demux/309 -> Jounce_Acceleration1/1  "L1"
  Demux/310 -> Jounce_Acceleration1/2  "L2"
  Demux/311 -> Jounce_Acceleration1/3  "R1"
  Demux/312 -> Jounce_Acceleration1/4  "R2"
  Jounce_Rate1/1 -> Inerter/5  "Jounce_Rate"
  Demux/313 -> Jounce_Rate1/1  "L1"
  Demux/314 -> Jounce_Rate1/2  "L2"
  Demux/315 -> Jounce_Rate1/3  "R1"
  Demux/316 -> Jounce_Rate1/4  "R2"
  inl_ride_inerter_data/1 -> OutputBus/36  "inl_ride_inerter_data"
  Demux/317 -> inl_ride_inerter_data/1  "acceleration_front"
  Demux/318 -> inl_ride_inerter_data/2  "acceleration_rear"
  Demux/319 -> inl_ride_inerter_data/3  "displacement_front"
  Demux/320 -> inl_ride_inerter_data/4  "displacement_rear"
  Demux/321 -> inl_ride_inerter_data/5  "force_front"
  Demux/322 -> inl_ride_inerter_data/6  "force_rear"
  inr_ride_inerter_data/1 -> OutputBus/37  "inr_ride_inerter_data"
  Demux/323 -> inr_ride_inerter_data/1  "acceleration_front"
  Demux/324 -> inr_ride_inerter_data/2  "acceleration_rear"
  Demux/325 -> inr_ride_inerter_data/3  "displacement_front"
  Demux/326 -> inr_ride_inerter_data/4  "displacement_rear"
  Demux/327 -> inr_ride_inerter_data/5  "force_front"
  Demux/328 -> inr_ride_inerter_data/6  "force_rear"
  ins_inerter_data/1 -> OutputBus/38  "ins_inerter_data"
  Demux/329 -> ins_inerter_data/1  "acceleration_front"
  Demux/330 -> ins_inerter_data/2  "acceleration_rear"
  Demux/331 -> ins_inerter_data/3  "displacement_front"
  Demux/332 -> ins_inerter_data/4  "displacement_rear"
  Demux/333 -> ins_inerter_data/5  "force_at_wheel_front"
  Demux/334 -> ins_inerter_data/6  "force_at_wheel_rear"
  Demux/335 -> ins_inerter_data/7  "force_front"
  Demux/336 -> ins_inerter_data/8  "force_rear"
  Demux/337 -> ins_inerter_data/9  "velocity_front"
  Demux/338 -> ins_inerter_data/10  "velocity_rear"
  jfs_torsional_stiffness_data/1 -> OutputBus/39  "jfs_torsional_stiffness_data"
  Demux/339 -> jfs_torsional_stiffness_data/1  "AX_1"
  Demux/340 -> jfs_torsional_stiffness_data/2  "AY_1"
  Demux/341 -> jfs_torsional_stiffness_data/3  "AZ_1"
  Demux/342 -> jfs_torsional_stiffness_data/4  "FX_1"
  Demux/343 -> jfs_torsional_stiffness_data/5  "FY_1"
  Demux/344 -> jfs_torsional_stiffness_data/6  "FZ_1"
  Demux/345 -> jfs_torsional_stiffness_data/7  "TX_1"
  Demux/346 -> jfs_torsional_stiffness_data/8  "TY_1"
  Demux/347 -> jfs_torsional_stiffness_data/9  "TZ_1"
  Demux/348 -> jfs_torsional_stiffness_data/10  "X_1"
  Demux/349 -> jfs_torsional_stiffness_data/11  "Y_1"
  Demux/350 -> jfs_torsional_stiffness_data/12  "Z_1"
  Jounce_Bumper/1 -> OutputBus/40  "Jounce_Bumper"
  Force_At_Bumper/1 -> Jounce_Bumper/1  "Force_At_Bumper"
  Demux/351 -> Force_At_Bumper/1  "L1"
  Demux/352 -> Force_At_Bumper/2  "L2"
  Demux/353 -> Force_At_Bumper/3  "R1"
  Demux/354 -> Force_At_Bumper/4  "R2"
  Force_At_Wheel2/1 -> Jounce_Bumper/2  "Force_At_Wheel"
  Demux/355 -> Force_At_Wheel2/1  "L1"
  Demux/356 -> Force_At_Wheel2/2  "L2"
  Demux/357 -> Force_At_Wheel2/3  "R1"
  Demux/358 -> Force_At_Wheel2/4  "R2"
  Jounce2/1 -> Jounce_Bumper/3  "Jounce"
  Demux/359 -> Jounce2/1  "L1"
  Demux/360 -> Jounce2/2  "L2"
  Demux/361 -> Jounce2/3  "R1"
  Demux/362 -> Jounce2/4  "R2"
  Jounce_Rate2/1 -> Jounce_Bumper/4  "Jounce_Rate"
  Demux/363 -> Jounce_Rate2/1  "L1"
  Demux/364 -> Jounce_Rate2/2  "L2"
  Demux/365 -> Jounce_Rate2/3  "R1"
  Demux/366 -> Jounce_Rate2/4  "R2"
  nsl_ride_spring_data/1 -> OutputBus/41  "nsl_ride_spring_data"
  Demux/367 -> nsl_ride_spring_data/1  "displacement_front"
  Demux/368 -> nsl_ride_spring_data/2  "displacement_rear"
  Demux/369 -> nsl_ride_spring_data/3  "force_front"
  Demux/370 -> nsl_ride_spring_data/4  "force_rear"
  Demux/371 -> nsl_ride_spring_data/5  "velocity_front"
  Demux/372 -> nsl_ride_spring_data/6  "velocity_rear"
  nsr_ride_spring_data/1 -> OutputBus/42  "nsr_ride_spring_data"
  Demux/373 -> nsr_ride_spring_data/1  "displacement_front"
  Demux/374 -> nsr_ride_spring_data/2  "displacement_rear"
  Demux/375 -> nsr_ride_spring_data/3  "force_front"
  Demux/376 -> nsr_ride_spring_data/4  "force_rear"
  Demux/377 -> nsr_ride_spring_data/5  "velocity_front"
  Demux/378 -> nsr_ride_spring_data/6  "velocity_rear"
  nss_ride_spring_data/1 -> OutputBus/43  "nss_ride_spring_data"
  Demux/379 -> nss_ride_spring_data/1  "displacement_front"
  Demux/380 -> nss_ride_spring_data/2  "displacement_rear"
  Demux/381 -> nss_ride_spring_data/3  "force_at_wheel_front"
  Demux/382 -> nss_ride_spring_data/4  "force_at_wheel_rear"
  Demux/383 -> nss_ride_spring_data/5  "force_front"
  Demux/384 -> nss_ride_spring_data/6  "force_rear"
  Demux/385 -> nss_ride_spring_data/7  "PID_PH_At_Spring_front"
  Demux/386 -> nss_ride_spring_data/8  "PID_PH_At_Spring_rear"
  Demux/387 -> nss_ride_spring_data/9  "velocity_front"
  Demux/388 -> nss_ride_spring_data/10  "velocity_rear"
  Rebound_Bumper/1 -> OutputBus/44  "Rebound_Bumper"
  Force_At_Bumper1/1 -> Rebound_Bumper/1  "Force_At_Bumper"
  Demux/389 -> Force_At_Bumper1/1  "L1"
  Demux/390 -> Force_At_Bumper1/2  "L2"
  Demux/391 -> Force_At_Bumper1/3  "R1"
  Demux/392 -> Force_At_Bumper1/4  "R2"
  Force_At_Wheel3/1 -> Rebound_Bumper/2  "Force_At_Wheel"
  Demux/393 -> Force_At_Wheel3/1  "L1"
  Demux/394 -> Force_At_Wheel3/2  "L2"
  Demux/395 -> Force_At_Wheel3/3  "R1"
  Demux/396 -> Force_At_Wheel3/4  "R2"
  Jounce3/1 -> Rebound_Bumper/3  "Jounce"
  Demux/397 -> Jounce3/1  "L1"
  Demux/398 -> Jounce3/2  "L2"
  Demux/399 -> Jounce3/3  "R1"
  Demux/400 -> Jounce3/4  "R2"
  Jounce_Rate3/1 -> Rebound_Bumper/4  "Jounce_Rate"
  Demux/401 -> Jounce_Rate3/1  "L1"
  Demux/402 -> Jounce_Rate3/2  "L2"
  Demux/403 -> Jounce_Rate3/3  "R1"
  Demux/404 -> Jounce_Rate3/4  "R2"
  res_dmp_rebound_stop_data/1 -> OutputBus/45  "res_dmp_rebound_stop_data"
  Demux/405 -> res_dmp_rebound_stop_data/1  "displacement_front"
  Demux/406 -> res_dmp_rebound_stop_data/2  "displacement_rear"
  Demux/407 -> res_dmp_rebound_stop_data/3  "force_front"
  Demux/408 -> res_dmp_rebound_stop_data/4  "force_rear"
  Demux/409 -> res_dmp_rebound_stop_data/5  "velocity_front"
  Demux/410 -> res_dmp_rebound_stop_data/6  "velocity_rear"
  res_ins_rebound_stop_data/1 -> OutputBus/46  "res_ins_rebound_stop_data"
  Demux/411 -> res_ins_rebound_stop_data/1  "displacement_front"
  Demux/412 -> res_ins_rebound_stop_data/2  "displacement_rear"
  Demux/413 -> res_ins_rebound_stop_data/3  "force_front"
  Demux/414 -> res_ins_rebound_stop_data/4  "force_rear"
  Demux/415 -> res_ins_rebound_stop_data/5  "velocity_front"
  Demux/416 -> res_ins_rebound_stop_data/6  "velocity_rear"
  res_roll_dmp_rebound_stop_data/1 -> OutputBus/47  "res_roll_dmp_rebound_stop_data"
  Demux/417 -> res_roll_dmp_rebound_stop_data/1  "displacement_front"
  Demux/418 -> res_roll_dmp_rebound_stop_data/2  "displacement_rear"
  Demux/419 -> res_roll_dmp_rebound_stop_data/3  "force_front"
  Demux/420 -> res_roll_dmp_rebound_stop_data/4  "force_rear"
  Demux/421 -> res_roll_dmp_rebound_stop_data/5  "velocity_front"
  Demux/422 -> res_roll_dmp_rebound_stop_data/6  "velocity_rear"
  res_spr_rebound_stop_data/1 -> OutputBus/48  "res_spr_rebound_stop_data"
  Demux/423 -> res_spr_rebound_stop_data/1  "displacement_front"
  Demux/424 -> res_spr_rebound_stop_data/2  "displacement_rear"
  Demux/425 -> res_spr_rebound_stop_data/3  "force_front"
  Demux/426 -> res_spr_rebound_stop_data/4  "force_rear"
  Demux/427 -> res_spr_rebound_stop_data/5  "velocity_front"
  Demux/428 -> res_spr_rebound_stop_data/6  "velocity_rear"
  rhl_front_setup_sensor_data/1 -> OutputBus/49  "rhl_front_setup_sensor_data"
  Demux/429 -> rhl_front_setup_sensor_data/1  "ride_height"
  rhl_rear_setup_sensor_data/1 -> OutputBus/50  "rhl_rear_setup_sensor_data"
  Demux/430 -> rhl_rear_setup_sensor_data/1  "ride_height"
  rhr_front_setup_sensor_data/1 -> OutputBus/51  "rhr_front_setup_sensor_data"
  Demux/431 -> rhr_front_setup_sensor_data/1  "ride_height"
  rhr_rear_setup_sensor_data/1 -> OutputBus/52  "rhr_rear_setup_sensor_data"
  Demux/432 -> rhr_rear_setup_sensor_data/1  "ride_height"
  rhs_front_setup_sensor_data/1 -> OutputBus/53  "rhs_front_setup_sensor_data"
  Demux/433 -> rhs_front_setup_sensor_data/1  "ride_height"
  rhs_rear_setup_sensor_data/1 -> OutputBus/54  "rhs_rear_setup_sensor_data"
  Demux/434 -> rhs_rear_setup_sensor_data/1  "ride_height"
  Road/1 -> OutputBus/55  "Road"
  Contact_Flag/1 -> Road/1  "Contact_Flag"
  Demux/435 -> Contact_Flag/1  "L1"
  Demux/436 -> Contact_Flag/2  "L2"
  Demux/437 -> Contact_Flag/3  "R1"
  Demux/438 -> Contact_Flag/4  "R2"
  Contact_Patch_Global_X/1 -> Road/2  "Contact_Patch_Global_X"
  Demux/439 -> Contact_Patch_Global_X/1  "L1"
  Demux/440 -> Contact_Patch_Global_X/2  "L2"
  Demux/441 -> Contact_Patch_Global_X/3  "R1"
  Demux/442 -> Contact_Patch_Global_X/4  "R2"
  Contact_Patch_Global_Y/1 -> Road/3  "Contact_Patch_Global_Y"
  Demux/443 -> Contact_Patch_Global_Y/1  "L1"
  Demux/444 -> Contact_Patch_Global_Y/2  "L2"
  Demux/445 -> Contact_Patch_Global_Y/3  "R1"
  Demux/446 -> Contact_Patch_Global_Y/4  "R2"
  Contact_Patch_Global_Z/1 -> Road/4  "Contact_Patch_Global_Z"
  Demux/447 -> Contact_Patch_Global_Z/1  "L1"
  Demux/448 -> Contact_Patch_Global_Z/2  "L2"
  Demux/449 -> Contact_Patch_Global_Z/3  "R1"
  Demux/450 -> Contact_Patch_Global_Z/4  "R2"
  Off_Road_Flag/1 -> Road/5  "Off_Road_Flag"
  Demux/451 -> Off_Road_Flag/1  "L1"
  Demux/452 -> Off_Road_Flag/2  "L2"
  Demux/453 -> Off_Road_Flag/3  "R1"
  Demux/454 -> Off_Road_Flag/4  "R2"
  Sensor/1 -> OutputBus/56  "Sensor"
  Demux/455 -> Sensor/1  "AccX_gyro"
  Demux/456 -> Sensor/2  "AccY_gyro"
  Demux/457 -> Sensor/3  "Ax"
  Demux/458 -> Sensor/4  "Ax_Without_Gravity"
  Demux/459 -> Sensor/5  "Ay"
  Demux/460 -> Sensor/6  "Ay_Without_Gravity"
  Demux/461 -> Sensor/7  "Az"
  Demux/462 -> Sensor/8  "Az_Without_Gravity"
  Demux/463 -> Sensor/9  "Global_X"
  Demux/464 -> Sensor/10  "Global_Y"
  Demux/465 -> Sensor/11  "Global_Z"
  Demux/466 -> Sensor/12  "Vx"
  Demux/467 -> Sensor/13  "Vx_gyro"
  Demux/468 -> Sensor/14  "Vy"
  Demux/469 -> Sensor/15  "Vz"
  Demux/470 -> Sensor/16  "YawRate_gyro"
  Spring/1 -> OutputBus/57  "Spring"
  Aggregate_Force_At_Wheel/1 -> Spring/1  "Aggregate_Force_At_Wheel"
  Demux/471 -> Aggregate_Force_At_Wheel/1  "L1"
  Demux/472 -> Aggregate_Force_At_Wheel/2  "L2"
  Demux/473 -> Aggregate_Force_At_Wheel/3  "R1"
  Demux/474 -> Aggregate_Force_At_Wheel/4  "R2"
  Force_At_Spring/1 -> Spring/2  "Force_At_Spring"
  Demux/475 -> Force_At_Spring/1  "L1"
  Demux/476 -> Force_At_Spring/2  "L2"
  Demux/477 -> Force_At_Spring/3  "R1"
  Demux/478 -> Force_At_Spring/4  "R2"
  Force_At_Wheel4/1 -> Spring/3  "Force_At_Wheel"
  Demux/479 -> Force_At_Wheel4/1  "L1"
  Demux/480 -> Force_At_Wheel4/2  "L2"
  Demux/481 -> Force_At_Wheel4/3  "R1"
  Demux/482 -> Force_At_Wheel4/4  "R2"
  Force_Aux_At_Wheel/1 -> Spring/4  "Force_Aux_At_Wheel"
  Demux/483 -> Force_Aux_At_Wheel/1  "L1"
  Demux/484 -> Force_Aux_At_Wheel/2  "L2"
  Demux/485 -> Force_Aux_At_Wheel/3  "R1"
  Demux/486 -> Force_Aux_At_Wheel/4  "R2"
  Jounce4/1 -> Spring/5  "Jounce"
  Demux/487 -> Jounce4/1  "L1"
  Demux/488 -> Jounce4/2  "L2"
  Demux/489 -> Jounce4/3  "R1"
  Demux/490 -> Jounce4/4  "R2"
  Jounce_Acceleration2/1 -> Spring/6  "Jounce_Acceleration"
  Demux/491 -> Jounce_Acceleration2/1  "L1"
  Demux/492 -> Jounce_Acceleration2/2  "L2"
  Demux/493 -> Jounce_Acceleration2/3  "R1"
  Demux/494 -> Jounce_Acceleration2/4  "R2"
  Jounce_Rate4/1 -> Spring/7  "Jounce_Rate"
  Demux/495 -> Jounce_Rate4/1  "L1"
  Demux/496 -> Jounce_Rate4/2  "L2"
  Demux/497 -> Jounce_Rate4/3  "R1"
  Demux/498 -> Jounce_Rate4/4  "R2"
  PID_CW_At_Spring/1 -> Spring/8  "PID_CW_At_Spring"
  Demux/499 -> PID_CW_At_Spring/1  "L1"
  Demux/500 -> PID_CW_At_Spring/2  "L2"
  Demux/501 -> PID_CW_At_Spring/3  "R1"
  Demux/502 -> PID_CW_At_Spring/4  "R2"
  PID_PH_At_Spring/1 -> Spring/9  "PID_PH_At_Spring"
  Demux/503 -> PID_PH_At_Spring/1  "L1"
  Demux/504 -> PID_PH_At_Spring/2  "L2"
  Demux/505 -> PID_PH_At_Spring/3  "R1"
  Demux/506 -> PID_PH_At_Spring/4  "R2"
  PID_RH_At_Spring/1 -> Spring/10  "PID_RH_At_Spring"
  Demux/507 -> PID_RH_At_Spring/1  "L1"
  Demux/508 -> PID_RH_At_Spring/2  "L2"
  Demux/509 -> PID_RH_At_Spring/3  "R1"
  Demux/510 -> PID_RH_At_Spring/4  "R2"
  Steering_System/1 -> OutputBus/58  "Steering_System"
  Demux/511 -> Steering_System/1  "DriveSim_Steering_Feedback_Torque"
  Demux/512 -> Steering_System/2  "Rack_displacement"
  Demux/513 -> Steering_System/3  "Rack_Force"
  Demux/514 -> Steering_System/4  "Steering_column_deformation"
  Demux/515 -> Steering_System/5  "Steering_Wheel_Torque"
  TieRod_Force_Left/1 -> Steering_System/6  "TieRod_Force_Left"
  Demux/516 -> TieRod_Force_Left/1  "X"
  Demux/517 -> TieRod_Force_Left/2  "Y"
  Demux/518 -> TieRod_Force_Left/3  "Z"
  TieRod_Force_Right/1 -> Steering_System/7  "TieRod_Force_Right"
  Demux/519 -> TieRod_Force_Right/1  "X"
  Demux/520 -> TieRod_Force_Right/2  "Y"
  Demux/521 -> TieRod_Force_Right/3  "Z"
  Demux/1284 -> Steering_System/8  "selected_eps_map"
  Demux/1285 -> Steering_System/9  "eccentricity_torque"
  Demux/1287 -> Steering_System/10  "pitman_arm_rotation"
  Demux/1288 -> Steering_System/11  "pitman_arm_saturated_rotation"
  Demux/1289 -> Steering_System/12  "pitman_arm_velocity"
  Demux/1290 -> Steering_System/13  "pitman_arm_acceleration"
  Suspension/1 -> OutputBus/59  "Suspension"
  Auxiliary_Roll_deformation_at_element/1 -> Suspension/1  "Auxiliary_Roll_deformation_at_element"
  Demux/522 -> Auxiliary_Roll_deformation_at_element/1  "SUSP1"
  Demux/523 -> Auxiliary_Roll_deformation_at_element/2  "SUSP2"
  Auxiliary_Roll_Force/1 -> Suspension/2  "Auxiliary_Roll_Force"
  Demux/524 -> Auxiliary_Roll_Force/1  "SUSP_L1"
  Demux/525 -> Auxiliary_Roll_Force/2  "SUSP_L2"
  Demux/526 -> Auxiliary_Roll_Force/3  "SUSP_R1"
  Demux/527 -> Auxiliary_Roll_Force/4  "SUSP_R2"
  Auxiliary_Roll_Force_at_element/1 -> Suspension/3  "Auxiliary_Roll_Force_at_element"
  Demux/528 -> Auxiliary_Roll_Force_at_element/1  "SUSP1"
  Demux/529 -> Auxiliary_Roll_Force_at_element/2  "SUSP2"
  base_acceleration/1 -> Suspension/4  "base_acceleration"
  Demux/530 -> base_acceleration/1  "L1"
  Demux/531 -> base_acceleration/2  "L2"
  Demux/532 -> base_acceleration/3  "R1"
  Demux/533 -> base_acceleration/4  "R2"
  base_deformation/1 -> Suspension/5  "base_deformation"
  Demux/534 -> base_deformation/1  "L1"
  Demux/535 -> base_deformation/2  "L2"
  Demux/536 -> base_deformation/3  "R1"
  Demux/537 -> base_deformation/4  "R2"
  base_velocity/1 -> Suspension/6  "base_velocity"
  Demux/538 -> base_velocity/1  "L1"
  Demux/539 -> base_velocity/2  "L2"
  Demux/540 -> base_velocity/3  "R1"
  Demux/541 -> base_velocity/4  "R2"
  Inst_Stiff_Deflection/1 -> Suspension/7  "Inst_Stiff_Deflection"
  Demux/542 -> Inst_Stiff_Deflection/1  "front_left"
  Demux/543 -> Inst_Stiff_Deflection/2  "front_right"
  Demux/544 -> Inst_Stiff_Deflection/3  "rear_left"
  Demux/545 -> Inst_Stiff_Deflection/4  "rear_right"
  Inst_Stiff_Force/1 -> Suspension/8  "Inst_Stiff_Force"
  Demux/546 -> Inst_Stiff_Force/1  "front_left"
  Demux/547 -> Inst_Stiff_Force/2  "front_right"
  Demux/548 -> Inst_Stiff_Force/3  "rear_left"
  Demux/549 -> Inst_Stiff_Force/4  "rear_right"
  Jounce5/1 -> Suspension/9  "Jounce"
  Demux/550 -> Jounce5/1  "L1"
  Demux/551 -> Jounce5/2  "L2"
  Demux/552 -> Jounce5/3  "R1"
  Demux/553 -> Jounce5/4  "R2"
  Jounce_Acceleration3/1 -> Suspension/10  "Jounce_Acceleration"
  Demux/554 -> Jounce_Acceleration3/1  "L1"
  Demux/555 -> Jounce_Acceleration3/2  "L2"
  Demux/556 -> Jounce_Acceleration3/3  "R1"
  Demux/557 -> Jounce_Acceleration3/4  "R2"
  Jounce_Rate5/1 -> Suspension/11  "Jounce_Rate"
  Demux/558 -> Jounce_Rate5/1  "L1"
  Demux/559 -> Jounce_Rate5/2  "L2"
  Demux/560 -> Jounce_Rate5/3  "R1"
  Demux/561 -> Jounce_Rate5/4  "R2"
  Kingpin_Moment/1 -> Suspension/12  "Kingpin_Moment"
  Demux/562 -> Kingpin_Moment/1  "SUSP1"
  Roll/1 -> Suspension/13  "Roll"
  Demux/563 -> Roll/1  "SUSP1"
  Demux/564 -> Roll/2  "SUSP2"
  Roll_Center_Height/1 -> Suspension/14  "Roll_Center_Height"
  Demux/565 -> Roll_Center_Height/1  "front"
  Demux/566 -> Roll_Center_Height/2  "rear"
  Roll_Center_Lateral_Displacement/1 -> Suspension/15  "Roll_Center_Lateral_Displacement"
  Demux/567 -> Roll_Center_Lateral_Displacement/1  "front"
  Demux/568 -> Roll_Center_Lateral_Displacement/2  "rear"
  Steering_Instant_Axis_Rotation/1 -> Suspension/16  "Steering_Instant_Axis_Rotation"
  Demux/569 -> Steering_Instant_Axis_Rotation/1  "L1"
  Demux/570 -> Steering_Instant_Axis_Rotation/2  "R1"
  System/1 -> OutputBus/60  "System"
  Demux/571 -> System/1  "Angular_Acceleration_Norm"
  Demux/572 -> System/2  "Angular_Speed_Norm"
  Demux/573 -> System/3  "Testrig_MMM_Fx"
  Demux/574 -> System/4  "Testrig_MMM_Fy"
  Demux/575 -> System/5  "Testrig_MMM_Mz"
  Demux/576 -> System/6  "Testrig_MMM_xd"
  Demux/577 -> System/7  "Testrig_MMM_xi"
  Demux/578 -> System/8  "Testrig_MMM_xp"
  Demux/579 -> System/9  "Testrig_MMM_yawd"
  Demux/580 -> System/10  "Testrig_MMM_yawi"
  Demux/581 -> System/11  "Testrig_MMM_yawp"
  Demux/582 -> System/12  "Testrig_MMM_yd"
  Demux/583 -> System/13  "Testrig_MMM_yi"
  Demux/584 -> System/14  "Testrig_MMM_yp"
  Demux/585 -> System/15  "Time"
  Demux/586 -> System/16  "Translational_Acceleration_Norm"
  Demux/587 -> System/17  "Translational_Speed_Norm"
  Demux/1301 -> System/18  "Solver_Status"
  System_Mass_Center/1 -> OutputBus/61  "System_Mass_Center"
  Demux/588 -> System_Mass_Center/1  "Global_Ax"
  Demux/589 -> System_Mass_Center/2  "Global_Ay"
  Demux/590 -> System_Mass_Center/3  "Global_Az"
  Demux/591 -> System_Mass_Center/4  "Global_Vx"
  Demux/592 -> System_Mass_Center/5  "Global_Vy"
  Demux/593 -> System_Mass_Center/6  "Global_Vz"
  Demux/594 -> System_Mass_Center/7  "Global_X"
  Demux/595 -> System_Mass_Center/8  "Global_Y"
  Demux/596 -> System_Mass_Center/9  "Global_Z"
  Demux/597 -> System_Mass_Center/10  "Normal_Acceleration"
  Demux/598 -> System_Mass_Center/11  "Path_Curvature"
  Demux/599 -> System_Mass_Center/12  "Speed"
  Demux/600 -> System_Mass_Center/13  "Tangential_Acceleration"
  til_wheel_tire_forces/1 -> OutputBus/62  "til_wheel_tire_forces"
  Demux/601 -> til_wheel_tire_forces/1  "aligning_torque_front"
  Demux/602 -> til_wheel_tire_forces/2  "aligning_torque_rear"
  Demux/603 -> til_wheel_tire_forces/3  "aligning_torque_twin_rear"
  Demux/604 -> til_wheel_tire_forces/4  "lateral_front"
  Demux/605 -> til_wheel_tire_forces/5  "lateral_rear"
  Demux/606 -> til_wheel_tire_forces/6  "lateral_twin_rear"
  Demux/607 -> til_wheel_tire_forces/7  "longitudinal_front"
  Demux/608 -> til_wheel_tire_forces/8  "longitudinal_rear"
  Demux/609 -> til_wheel_tire_forces/9  "longitudinal_twin_rear"
  Demux/610 -> til_wheel_tire_forces/10  "normal_front"
  Demux/611 -> til_wheel_tire_forces/11  "normal_rear"
  Demux/612 -> til_wheel_tire_forces/12  "normal_twin_rear"
  Demux/613 -> til_wheel_tire_forces/13  "overturning_moment_front"
  Demux/614 -> til_wheel_tire_forces/14  "overturning_moment_rear"
  Demux/615 -> til_wheel_tire_forces/15  "overturning_moment_twin_rear"
  Demux/616 -> til_wheel_tire_forces/16  "rolling_resistance_front"
  Demux/617 -> til_wheel_tire_forces/17  "rolling_resistance_rear"
  Demux/618 -> til_wheel_tire_forces/18  "rolling_resistance_twin_rear"
  til_wheel_tire_kinematics/1 -> OutputBus/63  "til_wheel_tire_kinematics"
  Demux/619 -> til_wheel_tire_kinematics/1  "inclination_angle_front"
  Demux/620 -> til_wheel_tire_kinematics/2  "inclination_angle_rear"
  Demux/621 -> til_wheel_tire_kinematics/3  "inclination_angle_twin_rear"
  Demux/622 -> til_wheel_tire_kinematics/4  "lateral_slip_front"
  Demux/623 -> til_wheel_tire_kinematics/5  "lateral_slip_rear"
  Demux/624 -> til_wheel_tire_kinematics/6  "lateral_slip_twin_rear"
  Demux/625 -> til_wheel_tire_kinematics/7  "longitudinal_slip_front"
  Demux/626 -> til_wheel_tire_kinematics/8  "longitudinal_slip_rear"
  Demux/627 -> til_wheel_tire_kinematics/9  "longitudinal_slip_twin_rear"
  til_wheel_tire_rolling_states/1 -> OutputBus/64  "til_wheel_tire_rolling_states"
  Demux/628 -> til_wheel_tire_rolling_states/1  "omega_actual_front"
  Demux/629 -> til_wheel_tire_rolling_states/2  "omega_actual_rear"
  Demux/630 -> til_wheel_tire_rolling_states/3  "omega_actual_twin_rear"
  Demux/631 -> til_wheel_tire_rolling_states/4  "omega_free_front"
  Demux/632 -> til_wheel_tire_rolling_states/5  "omega_free_rear"
  Demux/633 -> til_wheel_tire_rolling_states/6  "omega_free_twin_rear"
  Demux/634 -> til_wheel_tire_rolling_states/7  "rolling_radius_front"
  Demux/635 -> til_wheel_tire_rolling_states/8  "rolling_radius_rear"
  Demux/636 -> til_wheel_tire_rolling_states/9  "rolling_radius_twin_rear"
  Tire/1 -> OutputBus/65  "Tire"
  Actual_Tread_Speed/1 -> Tire/1  "Actual_Tread_Speed"
  Demux/637 -> Actual_Tread_Speed/1  "L1"
  Demux/638 -> Actual_Tread_Speed/2  "L2"
  Demux/639 -> Actual_Tread_Speed/3  "R1"
  Demux/640 -> Actual_Tread_Speed/4  "R2"
  Contact_Patch_Global_X1/1 -> Tire/2  "Contact_Patch_Global_X"
  Demux/641 -> Contact_Patch_Global_X1/1  "L1"
  Demux/642 -> Contact_Patch_Global_X1/2  "L2"
  Demux/643 -> Contact_Patch_Global_X1/3  "R1"
  Demux/644 -> Contact_Patch_Global_X1/4  "R2"
  Contact_Patch_Global_Y1/1 -> Tire/3  "Contact_Patch_Global_Y"
  Demux/645 -> Contact_Patch_Global_Y1/1  "L1"
  Demux/646 -> Contact_Patch_Global_Y1/2  "L2"
  Demux/647 -> Contact_Patch_Global_Y1/3  "R1"
  Demux/648 -> Contact_Patch_Global_Y1/4  "R2"
  Contact_Patch_Global_Z1/1 -> Tire/4  "Contact_Patch_Global_Z"
  Demux/649 -> Contact_Patch_Global_Z1/1  "L1"
  Demux/650 -> Contact_Patch_Global_Z1/2  "L2"
  Demux/651 -> Contact_Patch_Global_Z1/3  "R1"
  Demux/652 -> Contact_Patch_Global_Z1/4  "R2"
  Contact_Patch_Normal_X/1 -> Tire/5  "Contact_Patch_Normal_X"
  Demux/653 -> Contact_Patch_Normal_X/1  "L1"
  Demux/654 -> Contact_Patch_Normal_X/2  "L2"
  Demux/655 -> Contact_Patch_Normal_X/3  "R1"
  Demux/656 -> Contact_Patch_Normal_X/4  "R2"
  Contact_Patch_Normal_Y/1 -> Tire/6  "Contact_Patch_Normal_Y"
  Demux/657 -> Contact_Patch_Normal_Y/1  "L1"
  Demux/658 -> Contact_Patch_Normal_Y/2  "L2"
  Demux/659 -> Contact_Patch_Normal_Y/3  "R1"
  Demux/660 -> Contact_Patch_Normal_Y/4  "R2"
  Contact_Patch_Normal_Z/1 -> Tire/7  "Contact_Patch_Normal_Z"
  Demux/661 -> Contact_Patch_Normal_Z/1  "L1"
  Demux/662 -> Contact_Patch_Normal_Z/2  "L2"
  Demux/663 -> Contact_Patch_Normal_Z/3  "R1"
  Demux/664 -> Contact_Patch_Normal_Z/4  "R2"
  Effective_Closing_Speed/1 -> Tire/8  "Effective_Closing_Speed"
  Demux/665 -> Effective_Closing_Speed/1  "L1"
  Demux/666 -> Effective_Closing_Speed/2  "L2"
  Demux/667 -> Effective_Closing_Speed/3  "R1"
  Demux/668 -> Effective_Closing_Speed/4  "R2"
  Effective_Penetration/1 -> Tire/9  "Effective_Penetration"
  Demux/669 -> Effective_Penetration/1  "L1"
  Demux/670 -> Effective_Penetration/2  "L2"
  Demux/671 -> Effective_Penetration/3  "R1"
  Demux/672 -> Effective_Penetration/4  "R2"
  Effective_Rolling_Radius/1 -> Tire/10  "Effective_Rolling_Radius"
  Demux/673 -> Effective_Rolling_Radius/1  "L1"
  Demux/674 -> Effective_Rolling_Radius/2  "L2"
  Demux/675 -> Effective_Rolling_Radius/3  "R1"
  Demux/676 -> Effective_Rolling_Radius/4  "R2"
  Equivalent_Tread_Speed/1 -> Tire/11  "Equivalent_Tread_Speed"
  Demux/677 -> Equivalent_Tread_Speed/1  "L1"
  Demux/678 -> Equivalent_Tread_Speed/2  "L2"
  Demux/679 -> Equivalent_Tread_Speed/3  "R1"
  Demux/680 -> Equivalent_Tread_Speed/4  "R2"
  External_Friction_Scale_Factor/1 -> Tire/12  "External_Friction_Scale_Factor"
  Demux/681 -> External_Friction_Scale_Factor/1  "L1"
  Demux/682 -> External_Friction_Scale_Factor/2  "L2"
  Demux/683 -> External_Friction_Scale_Factor/3  "R1"
  Demux/684 -> External_Friction_Scale_Factor/4  "R2"
  Ground_Surface_Contact_Patch_Vx/1 -> Tire/13  "Ground_Surface_Contact_Patch_Vx"
  Demux/685 -> Ground_Surface_Contact_Patch_Vx/1  "L1"
  Demux/686 -> Ground_Surface_Contact_Patch_Vx/2  "L2"
  Demux/687 -> Ground_Surface_Contact_Patch_Vx/3  "R1"
  Demux/688 -> Ground_Surface_Contact_Patch_Vx/4  "R2"
  Ground_Surface_Contact_Patch_Vy/1 -> Tire/14  "Ground_Surface_Contact_Patch_Vy"
  Demux/689 -> Ground_Surface_Contact_Patch_Vy/1  "L1"
  Demux/690 -> Ground_Surface_Contact_Patch_Vy/2  "L2"
  Demux/691 -> Ground_Surface_Contact_Patch_Vy/3  "R1"
  Demux/692 -> Ground_Surface_Contact_Patch_Vy/4  "R2"
  Ground_Surface_Force_X/1 -> Tire/15  "Ground_Surface_Force_X"
  Demux/693 -> Ground_Surface_Force_X/1  "L1"
  Demux/694 -> Ground_Surface_Force_X/2  "L2"
  Demux/695 -> Ground_Surface_Force_X/3  "R1"
  Demux/696 -> Ground_Surface_Force_X/4  "R2"
  Ground_Surface_Force_Y/1 -> Tire/16  "Ground_Surface_Force_Y"
  Demux/697 -> Ground_Surface_Force_Y/1  "L1"
  Demux/698 -> Ground_Surface_Force_Y/2  "L2"
  Demux/699 -> Ground_Surface_Force_Y/3  "R1"
  Demux/700 -> Ground_Surface_Force_Y/4  "R2"
  Ground_Surface_Force_Z/1 -> Tire/17  "Ground_Surface_Force_Z"
  Demux/701 -> Ground_Surface_Force_Z/1  "L1"
  Demux/702 -> Ground_Surface_Force_Z/2  "L2"
  Demux/703 -> Ground_Surface_Force_Z/3  "R1"
  Demux/704 -> Ground_Surface_Force_Z/4  "R2"
  Ground_Surface_Gyroscopic_Moment/1 -> Tire/18  "Ground_Surface_Gyroscopic_Moment"
  Demux/705 -> Ground_Surface_Gyroscopic_Moment/1  "L1"
  Demux/706 -> Ground_Surface_Gyroscopic_Moment/2  "L2"
  Demux/707 -> Ground_Surface_Gyroscopic_Moment/3  "R1"
  Demux/708 -> Ground_Surface_Gyroscopic_Moment/4  "R2"
  Ground_Surface_Kappa_Fy/1 -> Tire/19  "Ground_Surface_Kappa_Fy"
  Demux/709 -> Ground_Surface_Kappa_Fy/1  "L1"
  Demux/710 -> Ground_Surface_Kappa_Fy/2  "L2"
  Demux/711 -> Ground_Surface_Kappa_Fy/3  "R1"
  Demux/712 -> Ground_Surface_Kappa_Fy/4  "R2"
  Ground_Surface_Moment_X/1 -> Tire/20  "Ground_Surface_Moment_X"
  Demux/713 -> Ground_Surface_Moment_X/1  "L1"
  Demux/714 -> Ground_Surface_Moment_X/2  "L2"
  Demux/715 -> Ground_Surface_Moment_X/3  "R1"
  Demux/716 -> Ground_Surface_Moment_X/4  "R2"
  Ground_Surface_Moment_Y/1 -> Tire/21  "Ground_Surface_Moment_Y"
  Demux/717 -> Ground_Surface_Moment_Y/1  "L1"
  Demux/718 -> Ground_Surface_Moment_Y/2  "L2"
  Demux/719 -> Ground_Surface_Moment_Y/3  "R1"
  Demux/720 -> Ground_Surface_Moment_Y/4  "R2"
  Ground_Surface_Moment_Z/1 -> Tire/22  "Ground_Surface_Moment_Z"
  Demux/721 -> Ground_Surface_Moment_Z/1  "L1"
  Demux/722 -> Ground_Surface_Moment_Z/2  "L2"
  Demux/723 -> Ground_Surface_Moment_Z/3  "R1"
  Demux/724 -> Ground_Surface_Moment_Z/4  "R2"
  Ground_Surface_Peak_Friction_X/1 -> Tire/23  "Ground_Surface_Peak_Friction_X"
  Demux/725 -> Ground_Surface_Peak_Friction_X/1  "L1"
  Demux/726 -> Ground_Surface_Peak_Friction_X/2  "L2"
  Demux/727 -> Ground_Surface_Peak_Friction_X/3  "R1"
  Demux/728 -> Ground_Surface_Peak_Friction_X/4  "R2"
  Ground_Surface_Peak_Friction_Y/1 -> Tire/24  "Ground_Surface_Peak_Friction_Y"
  Demux/729 -> Ground_Surface_Peak_Friction_Y/1  "L1"
  Demux/730 -> Ground_Surface_Peak_Friction_Y/2  "L2"
  Demux/731 -> Ground_Surface_Peak_Friction_Y/3  "R1"
  Demux/732 -> Ground_Surface_Peak_Friction_Y/4  "R2"
  Ground_Surface_Residual_Torque/1 -> Tire/25  "Ground_Surface_Residual_Torque"
  Demux/733 -> Ground_Surface_Residual_Torque/1  "L1"
  Demux/734 -> Ground_Surface_Residual_Torque/2  "L2"
  Demux/735 -> Ground_Surface_Residual_Torque/3  "R1"
  Demux/736 -> Ground_Surface_Residual_Torque/4  "R2"
  Hub_Carrier_Force_Global_X/1 -> Tire/26  "Hub_Carrier_Force_Global_X"
  Demux/737 -> Hub_Carrier_Force_Global_X/1  "L1"
  Demux/738 -> Hub_Carrier_Force_Global_X/2  "L2"
  Demux/739 -> Hub_Carrier_Force_Global_X/3  "R1"
  Demux/740 -> Hub_Carrier_Force_Global_X/4  "R2"
  Hub_Carrier_Force_Global_Y/1 -> Tire/27  "Hub_Carrier_Force_Global_Y"
  Demux/741 -> Hub_Carrier_Force_Global_Y/1  "L1"
  Demux/742 -> Hub_Carrier_Force_Global_Y/2  "L2"
  Demux/743 -> Hub_Carrier_Force_Global_Y/3  "R1"
  Demux/744 -> Hub_Carrier_Force_Global_Y/4  "R2"
  Hub_Carrier_Force_Global_Z/1 -> Tire/28  "Hub_Carrier_Force_Global_Z"
  Demux/745 -> Hub_Carrier_Force_Global_Z/1  "L1"
  Demux/746 -> Hub_Carrier_Force_Global_Z/2  "L2"
  Demux/747 -> Hub_Carrier_Force_Global_Z/3  "R1"
  Demux/748 -> Hub_Carrier_Force_Global_Z/4  "R2"
  Hub_Carrier_Force_Local_X/1 -> Tire/29  "Hub_Carrier_Force_Local_X"
  Demux/749 -> Hub_Carrier_Force_Local_X/1  "L1"
  Demux/750 -> Hub_Carrier_Force_Local_X/2  "L2"
  Demux/751 -> Hub_Carrier_Force_Local_X/3  "R1"
  Demux/752 -> Hub_Carrier_Force_Local_X/4  "R2"
  Hub_Carrier_Force_Local_Y/1 -> Tire/30  "Hub_Carrier_Force_Local_Y"
  Demux/753 -> Hub_Carrier_Force_Local_Y/1  "L1"
  Demux/754 -> Hub_Carrier_Force_Local_Y/2  "L2"
  Demux/755 -> Hub_Carrier_Force_Local_Y/3  "R1"
  Demux/756 -> Hub_Carrier_Force_Local_Y/4  "R2"
  Hub_Carrier_Force_Local_Z/1 -> Tire/31  "Hub_Carrier_Force_Local_Z"
  Demux/757 -> Hub_Carrier_Force_Local_Z/1  "L1"
  Demux/758 -> Hub_Carrier_Force_Local_Z/2  "L2"
  Demux/759 -> Hub_Carrier_Force_Local_Z/3  "R1"
  Demux/760 -> Hub_Carrier_Force_Local_Z/4  "R2"
  Hub_Carrier_Moment_Global_X/1 -> Tire/32  "Hub_Carrier_Moment_Global_X"
  Demux/761 -> Hub_Carrier_Moment_Global_X/1  "L1"
  Demux/762 -> Hub_Carrier_Moment_Global_X/2  "L2"
  Demux/763 -> Hub_Carrier_Moment_Global_X/3  "R1"
  Demux/764 -> Hub_Carrier_Moment_Global_X/4  "R2"
  Hub_Carrier_Moment_Global_Y/1 -> Tire/33  "Hub_Carrier_Moment_Global_Y"
  Demux/765 -> Hub_Carrier_Moment_Global_Y/1  "L1"
  Demux/766 -> Hub_Carrier_Moment_Global_Y/2  "L2"
  Demux/767 -> Hub_Carrier_Moment_Global_Y/3  "R1"
  Demux/768 -> Hub_Carrier_Moment_Global_Y/4  "R2"
  Hub_Carrier_Moment_Global_Z/1 -> Tire/34  "Hub_Carrier_Moment_Global_Z"
  Demux/769 -> Hub_Carrier_Moment_Global_Z/1  "L1"
  Demux/770 -> Hub_Carrier_Moment_Global_Z/2  "L2"
  Demux/771 -> Hub_Carrier_Moment_Global_Z/3  "R1"
  Demux/772 -> Hub_Carrier_Moment_Global_Z/4  "R2"
  Hub_Carrier_Moment_Local_X/1 -> Tire/35  "Hub_Carrier_Moment_Local_X"
  Demux/773 -> Hub_Carrier_Moment_Local_X/1  "L1"
  Demux/774 -> Hub_Carrier_Moment_Local_X/2  "L2"
  Demux/775 -> Hub_Carrier_Moment_Local_X/3  "R1"
  Demux/776 -> Hub_Carrier_Moment_Local_X/4  "R2"
  Hub_Carrier_Moment_Local_Y/1 -> Tire/36  "Hub_Carrier_Moment_Local_Y"
  Demux/777 -> Hub_Carrier_Moment_Local_Y/1  "L1"
  Demux/778 -> Hub_Carrier_Moment_Local_Y/2  "L2"
  Demux/779 -> Hub_Carrier_Moment_Local_Y/3  "R1"
  Demux/780 -> Hub_Carrier_Moment_Local_Y/4  "R2"
  Hub_Carrier_Moment_Local_Z/1 -> Tire/37  "Hub_Carrier_Moment_Local_Z"
  Demux/781 -> Hub_Carrier_Moment_Local_Z/1  "L1"
  Demux/782 -> Hub_Carrier_Moment_Local_Z/2  "L2"
  Demux/783 -> Hub_Carrier_Moment_Local_Z/3  "R1"
  Demux/784 -> Hub_Carrier_Moment_Local_Z/4  "R2"
  Lateral_Relaxation_Length/1 -> Tire/38  "Lateral_Relaxation_Length"
  Demux/785 -> Lateral_Relaxation_Length/1  "L1"
  Demux/786 -> Lateral_Relaxation_Length/2  "L2"
  Demux/787 -> Lateral_Relaxation_Length/3  "R1"
  Demux/788 -> Lateral_Relaxation_Length/4  "R2"
  Lateral_Slip_Without_Lag/1 -> Tire/39  "Lateral_Slip_Without_Lag"
  Demux/789 -> Lateral_Slip_Without_Lag/1  "L1"
  Demux/790 -> Lateral_Slip_Without_Lag/2  "L2"
  Demux/791 -> Lateral_Slip_Without_Lag/3  "R1"
  Demux/792 -> Lateral_Slip_Without_Lag/4  "R2"
  Lateral_Slip_With_Lag/1 -> Tire/40  "Lateral_Slip_With_Lag"
  Demux/793 -> Lateral_Slip_With_Lag/1  "L1"
  Demux/794 -> Lateral_Slip_With_Lag/2  "L2"
  Demux/795 -> Lateral_Slip_With_Lag/3  "R1"
  Demux/796 -> Lateral_Slip_With_Lag/4  "R2"
  Loaded_Radius/1 -> Tire/41  "Loaded_Radius"
  Demux/797 -> Loaded_Radius/1  "L1"
  Demux/798 -> Loaded_Radius/2  "L2"
  Demux/799 -> Loaded_Radius/3  "R1"
  Demux/800 -> Loaded_Radius/4  "R2"
  Longitudinal_Relaxation_Length/1 -> Tire/42  "Longitudinal_Relaxation_Length"
  Demux/801 -> Longitudinal_Relaxation_Length/1  "L1"
  Demux/802 -> Longitudinal_Relaxation_Length/2  "L2"
  Demux/803 -> Longitudinal_Relaxation_Length/3  "R1"
  Demux/804 -> Longitudinal_Relaxation_Length/4  "R2"
  Longitudinal_Slip_Without_Lag/1 -> Tire/43  "Longitudinal_Slip_Without_Lag"
  Demux/805 -> Longitudinal_Slip_Without_Lag/1  "L1"
  Demux/806 -> Longitudinal_Slip_Without_Lag/2  "L2"
  Demux/807 -> Longitudinal_Slip_Without_Lag/3  "R1"
  Demux/808 -> Longitudinal_Slip_Without_Lag/4  "R2"
  Longitudinal_Slip_With_Lag/1 -> Tire/44  "Longitudinal_Slip_With_Lag"
  Demux/809 -> Longitudinal_Slip_With_Lag/1  "L1"
  Demux/810 -> Longitudinal_Slip_With_Lag/2  "L2"
  Demux/811 -> Longitudinal_Slip_With_Lag/3  "R1"
  Demux/812 -> Longitudinal_Slip_With_Lag/4  "R2"
  Moment_Arm_Of_Fx/1 -> Tire/45  "Moment_Arm_Of_Fx"
  Demux/813 -> Moment_Arm_Of_Fx/1  "L1"
  Demux/814 -> Moment_Arm_Of_Fx/2  "L2"
  Demux/815 -> Moment_Arm_Of_Fx/3  "R1"
  Demux/816 -> Moment_Arm_Of_Fx/4  "R2"
  Pneumatic_Trail/1 -> Tire/46  "Pneumatic_Trail"
  Demux/817 -> Pneumatic_Trail/1  "L1"
  Demux/818 -> Pneumatic_Trail/2  "L2"
  Demux/819 -> Pneumatic_Trail/3  "R1"
  Demux/820 -> Pneumatic_Trail/4  "R2"
  Pressure/1 -> Tire/47  "Pressure"
  Demux/821 -> Pressure/1  "L1"
  Demux/822 -> Pressure/2  "L2"
  Demux/823 -> Pressure/3  "R1"
  Demux/824 -> Pressure/4  "R2"
  Road_friction/1 -> Tire/48  "Road_friction"
  Demux/825 -> Road_friction/1  "L1"
  Demux/826 -> Road_friction/2  "L2"
  Demux/827 -> Road_friction/3  "R1"
  Demux/828 -> Road_friction/4  "R2"
  Temperature_1/1 -> Tire/49  "Temperature_1"
  Demux/829 -> Temperature_1/1  "L1"
  Demux/830 -> Temperature_1/2  "L2"
  Demux/831 -> Temperature_1/3  "R1"
  Demux/832 -> Temperature_1/4  "R2"
  Temperature_2/1 -> Tire/50  "Temperature_2"
  Demux/833 -> Temperature_2/1  "L1"
  Demux/834 -> Temperature_2/2  "L2"
  Demux/835 -> Temperature_2/3  "R1"
  Demux/836 -> Temperature_2/4  "R2"
  Temperature_3/1 -> Tire/51  "Temperature_3"
  Demux/837 -> Temperature_3/1  "L1"
  Demux/838 -> Temperature_3/2  "L2"
  Demux/839 -> Temperature_3/3  "R1"
  Demux/840 -> Temperature_3/4  "R2"
  Temperature_4/1 -> Tire/52  "Temperature_4"
  Demux/841 -> Temperature_4/1  "L1"
  Demux/842 -> Temperature_4/2  "L2"
  Demux/843 -> Temperature_4/3  "R1"
  Demux/844 -> Temperature_4/4  "R2"
  User_Input_Contact_Patch_Global_Z_Perturbation/1 -> Tire/53  "User_Input_Contact_Patch_Global_Z_Perturbation"
  Demux/845 -> User_Input_Contact_Patch_Global_Z_Perturbation/1  "L1"
  Demux/846 -> User_Input_Contact_Patch_Global_Z_Perturbation/2  "L2"
  Demux/847 -> User_Input_Contact_Patch_Global_Z_Perturbation/3  "R1"
  Demux/848 -> User_Input_Contact_Patch_Global_Z_Perturbation/4  "R2"
  Wear/1 -> Tire/54  "Wear"
  Demux/849 -> Wear/1  "L1"
  Demux/850 -> Wear/2  "L2"
  Demux/851 -> Wear/3  "R1"
  Demux/852 -> Wear/4  "R2"
  tir_wheel_tire_forces/1 -> OutputBus/66  "tir_wheel_tire_forces"
  Demux/853 -> tir_wheel_tire_forces/1  "aligning_torque_front"
  Demux/854 -> tir_wheel_tire_forces/2  "aligning_torque_rear"
  Demux/855 -> tir_wheel_tire_forces/3  "aligning_torque_twin_rear"
  Demux/856 -> tir_wheel_tire_forces/4  "lateral_front"
  Demux/857 -> tir_wheel_tire_forces/5  "lateral_rear"
  Demux/858 -> tir_wheel_tire_forces/6  "lateral_twin_rear"
  Demux/859 -> tir_wheel_tire_forces/7  "longitudinal_front"
  Demux/860 -> tir_wheel_tire_forces/8  "longitudinal_rear"
  Demux/861 -> tir_wheel_tire_forces/9  "longitudinal_twin_rear"
  Demux/862 -> tir_wheel_tire_forces/10  "normal_front"
  Demux/863 -> tir_wheel_tire_forces/11  "normal_rear"
  Demux/864 -> tir_wheel_tire_forces/12  "normal_twin_rear"
  Demux/865 -> tir_wheel_tire_forces/13  "overturning_moment_front"
  Demux/866 -> tir_wheel_tire_forces/14  "overturning_moment_rear"
  Demux/867 -> tir_wheel_tire_forces/15  "overturning_moment_twin_rear"
  Demux/868 -> tir_wheel_tire_forces/16  "rolling_resistance_front"
  Demux/869 -> tir_wheel_tire_forces/17  "rolling_resistance_rear"
  Demux/870 -> tir_wheel_tire_forces/18  "rolling_resistance_twin_rear"
  tir_wheel_tire_kinematics/1 -> OutputBus/67  "tir_wheel_tire_kinematics"
  Demux/871 -> tir_wheel_tire_kinematics/1  "inclination_angle_front"
  Demux/872 -> tir_wheel_tire_kinematics/2  "inclination_angle_rear"
  Demux/873 -> tir_wheel_tire_kinematics/3  "inclination_angle_twin_rear"
  Demux/874 -> tir_wheel_tire_kinematics/4  "lateral_slip_front"
  Demux/875 -> tir_wheel_tire_kinematics/5  "lateral_slip_rear"
  Demux/876 -> tir_wheel_tire_kinematics/6  "lateral_slip_twin_rear"
  Demux/877 -> tir_wheel_tire_kinematics/7  "longitudinal_slip_front"
  Demux/878 -> tir_wheel_tire_kinematics/8  "longitudinal_slip_rear"
  Demux/879 -> tir_wheel_tire_kinematics/9  "longitudinal_slip_twin_rear"
  tir_wheel_tire_rolling_states/1 -> OutputBus/68  "tir_wheel_tire_rolling_states"
  Demux/880 -> tir_wheel_tire_rolling_states/1  "omega_actual_front"
  Demux/881 -> tir_wheel_tire_rolling_states/2  "omega_actual_rear"
  Demux/882 -> tir_wheel_tire_rolling_states/3  "omega_actual_twin_rear"
  Demux/883 -> tir_wheel_tire_rolling_states/4  "omega_free_front"
  Demux/884 -> tir_wheel_tire_rolling_states/5  "omega_free_rear"
  Demux/885 -> tir_wheel_tire_rolling_states/6  "omega_free_twin_rear"
  Demux/886 -> tir_wheel_tire_rolling_states/7  "rolling_radius_front"
  Demux/887 -> tir_wheel_tire_rolling_states/8  "rolling_radius_rear"
  Demux/888 -> tir_wheel_tire_rolling_states/9  "rolling_radius_twin_rear"
  torque_converter/1 -> OutputBus/69  "torque_converter"
  Demux/889 -> torque_converter/1  "capacity_factor"
  Demux/890 -> torque_converter/2  "efficiency"
  Demux/891 -> torque_converter/3  "gearbox_inputshaft_alpha"
  Demux/892 -> torque_converter/4  "gearbox_inputshaft_angle"
  Demux/893 -> torque_converter/5  "gearbox_inputshaft_omega"
  Demux/894 -> torque_converter/6  "inputplate_torque"
  Demux/895 -> torque_converter/7  "speed_ratio"
  Demux/896 -> torque_converter/8  "torque"
  Demux/897 -> torque_converter/9  "torque_ratio"
  transmission/1 -> OutputBus/70  "transmission"
  Demux/898 -> transmission/1  "automatic_gearbox_shifting_mode"
  Demux/899 -> transmission/2  "clutch_outputplate_torque"
  Demux/900 -> transmission/3  "diff_central_inputshaft_alpha"
  Demux/901 -> transmission/4  "diff_central_inputshaft_angle"
  Demux/902 -> transmission/5  "diff_central_inputshaft_omega"
  Demux/903 -> transmission/6  "gear"
  Demux/904 -> transmission/7  "input_rpm"
  Demux/905 -> transmission/8  "output_rpm"
  Demux/906 -> transmission/9  "ratio"
  Demux/907 -> transmission/10  "torque"
  Demux/1292 -> transmission/11  "manual_shifting_activity"
  ues_third_spring_data/1 -> OutputBus/71  "ues_third_spring_data"
  Demux/908 -> ues_third_spring_data/1  "displacement_front"
  Demux/909 -> ues_third_spring_data/2  "displacement_rear"
  Demux/910 -> ues_third_spring_data/3  "force_front"
  Demux/911 -> ues_third_spring_data/4  "force_rear"
  Demux/912 -> ues_third_spring_data/5  "velocity_front"
  Demux/913 -> ues_third_spring_data/6  "velocity_rear"
  upright_accelerometer/1 -> OutputBus/72  "upright_accelerometer"
  Demux/914 -> upright_accelerometer/1  "Z_left_front"
  Demux/915 -> upright_accelerometer/2  "Z_left_rear"
  Demux/916 -> upright_accelerometer/3  "Z_right_front"
  Demux/917 -> upright_accelerometer/4  "Z_right_rear"
  Vehicle/1 -> OutputBus/73  "Vehicle"
  Demux/918 -> Vehicle/1  "Body_Fixed_Alpha_X"
  Demux/919 -> Vehicle/2  "Body_Fixed_Alpha_Y"
  Demux/920 -> Vehicle/3  "Body_Fixed_Alpha_Z"
  Demux/921 -> Vehicle/4  "Body_Fixed_Omega_X"
  Demux/922 -> Vehicle/5  "Body_Fixed_Omega_Y"
  Demux/923 -> Vehicle/6  "Body_Fixed_Omega_Z"
  Demux/924 -> Vehicle/7  "CM_Body_Fixed_Ax"
  Demux/925 -> Vehicle/8  "CM_Body_Fixed_Ay"
  Demux/926 -> Vehicle/9  "CM_Body_Fixed_Az"
  Demux/927 -> Vehicle/10  "CM_Body_Fixed_Vx"
  Demux/928 -> Vehicle/11  "CM_Body_Fixed_Vy"
  Demux/929 -> Vehicle/12  "CM_Body_Fixed_Vz"
  Demux/930 -> Vehicle/13  "CM_Global_And_Tracking_Az"
  Demux/931 -> Vehicle/14  "CM_Global_And_Tracking_Vz"
  Demux/932 -> Vehicle/15  "CM_Global_Ax"
  Demux/933 -> Vehicle/16  "CM_Global_Ay"
  Demux/934 -> Vehicle/17  "CM_Global_Vx"
  Demux/935 -> Vehicle/18  "CM_Global_Vy"
  Demux/936 -> Vehicle/19  "CM_Global_X"
  Demux/937 -> Vehicle/20  "CM_Global_Y"
  Demux/938 -> Vehicle/21  "CM_Global_Z"
  Demux/939 -> Vehicle/22  "CM_Tracking_Ax"
  Demux/940 -> Vehicle/23  "CM_Tracking_Ay"
  Demux/941 -> Vehicle/24  "CM_Tracking_Vx"
  Demux/942 -> Vehicle/25  "CM_Tracking_Vy"
  Demux/943 -> Vehicle/26  "cross_weight_PID"
  Demux/944 -> Vehicle/27  "Euler_Roll"
  Demux/945 -> Vehicle/28  "front_ride_height_at_center_point"
  Demux/946 -> Vehicle/29  "Global_Alpha_X"
  Demux/947 -> Vehicle/30  "Global_Alpha_Y"
  Demux/948 -> Vehicle/31  "Global_Alpha_Z"
  Demux/949 -> Vehicle/32  "Global_Omega_X"
  Demux/950 -> Vehicle/33  "Global_Omega_Y"
  Demux/951 -> Vehicle/34  "Global_Omega_Z"
  Demux/952 -> Vehicle/35  "Inclination_Roll"
  Demux/953 -> Vehicle/36  "Origin_Distance_Traveled"
  Demux/954 -> Vehicle/37  "Origin_Global_X"
  Demux/955 -> Vehicle/38  "Origin_Global_Y"
  Demux/956 -> Vehicle/39  "Origin_Global_Z"
  Demux/957 -> Vehicle/40  "Origin_Global_Z_wrt_road_mk"
  Demux/958 -> Vehicle/41  "Pitch"
  Demux/959 -> Vehicle/42  "Side_Slip_Angle"
  Demux/960 -> Vehicle/43  "Side_Slip_Angle_Rate"
  Demux/961 -> Vehicle/44  "Understeer_Gradient"
  Demux/962 -> Vehicle/45  "Understeer_Stability_Factor"
  Demux/963 -> Vehicle/46  "Yaw"
  Vehicle_States/1 -> OutputBus/74  "Vehicle_States"
  Demux/964 -> Vehicle_States/1  "horizontal_vel_wrt_road"
  Demux/965 -> Vehicle_States/2  "lateral_acc_wrt_road"
  Demux/966 -> Vehicle_States/3  "lateral_disp"
  Demux/967 -> Vehicle_States/4  "lateral_vel_wrt_road"
  Demux/968 -> Vehicle_States/5  "longitudinal_acc_wrt_road"
  Demux/969 -> Vehicle_States/6  "longitudinal_disp"
  Demux/970 -> Vehicle_States/7  "longitudinal_vel_wrt_road"
  Demux/971 -> Vehicle_States/8  "pitch_angle"
  Demux/972 -> Vehicle_States/9  "pitch_angular_acc_wrt_road"
  Demux/973 -> Vehicle_States/10  "pitch_angular_vel_wrt_road"
  Demux/974 -> Vehicle_States/11  "roll_angle"
  Demux/975 -> Vehicle_States/12  "roll_angular_acc_wrt_road"
  Demux/976 -> Vehicle_States/13  "roll_angular_vel_wrt_road"
  Demux/977 -> Vehicle_States/14  "side_slip"
  Demux/978 -> Vehicle_States/15  "vertical_acc_wrt_road"
  Demux/979 -> Vehicle_States/16  "vertical_disp"
  Demux/980 -> Vehicle_States/17  "vertical_vel_wrt_road"
  Demux/981 -> Vehicle_States/18  "yaw_angle"
  Demux/982 -> Vehicle_States/19  "yaw_angular_acc_wrt_road"
  Demux/983 -> Vehicle_States/20  "yaw_angular_vel_wrt_road"
  Wheel/1 -> OutputBus/75  "Wheel"
  Alpha/1 -> Wheel/1  "Alpha"
  Demux/984 -> Alpha/1  "L1"
  Demux/985 -> Alpha/2  "L2"
  Demux/986 -> Alpha/3  "R1"
  Demux/987 -> Alpha/4  "R2"
  Caster_Angle/1 -> Wheel/2  "Caster_Angle"
  Demux/988 -> Caster_Angle/1  "left"
  Demux/989 -> Caster_Angle/2  "right"
  Drive_Moment/1 -> Wheel/3  "Drive_Moment"
  Demux/990 -> Drive_Moment/1  "L1"
  Demux/991 -> Drive_Moment/2  "L2"
  Demux/992 -> Drive_Moment/3  "R1"
  Demux/993 -> Drive_Moment/4  "R2"
  Euler_Roll/1 -> Wheel/4  "Euler_Roll"
  Demux/994 -> Euler_Roll/1  "L1"
  Demux/995 -> Euler_Roll/2  "L2"
  Demux/996 -> Euler_Roll/3  "R1"
  Demux/997 -> Euler_Roll/4  "R2"
  Global_Omega_X/1 -> Wheel/5  "Global_Omega_X"
  Demux/998 -> Global_Omega_X/1  "L1"
  Demux/999 -> Global_Omega_X/2  "L2"
  Demux/1000 -> Global_Omega_X/3  "R1"
  Demux/1001 -> Global_Omega_X/4  "R2"
  Global_Omega_Y/1 -> Wheel/6  "Global_Omega_Y"
  Demux/1002 -> Global_Omega_Y/1  "L1"
  Demux/1003 -> Global_Omega_Y/2  "L2"
  Demux/1004 -> Global_Omega_Y/3  "R1"
  Demux/1005 -> Global_Omega_Y/4  "R2"
  Global_Omega_Z/1 -> Wheel/7  "Global_Omega_Z"
  Demux/1006 -> Global_Omega_Z/1  "L1"
  Demux/1007 -> Global_Omega_Z/2  "L2"
  Demux/1008 -> Global_Omega_Z/3  "R1"
  Demux/1009 -> Global_Omega_Z/4  "R2"
  Global_Vx/1 -> Wheel/8  "Global_Vx"
  Demux/1010 -> Global_Vx/1  "L1"
  Demux/1011 -> Global_Vx/2  "L2"
  Demux/1012 -> Global_Vx/3  "R1"
  Demux/1013 -> Global_Vx/4  "R2"
  Global_Vy/1 -> Wheel/9  "Global_Vy"
  Demux/1014 -> Global_Vy/1  "L1"
  Demux/1015 -> Global_Vy/2  "L2"
  Demux/1016 -> Global_Vy/3  "R1"
  Demux/1017 -> Global_Vy/4  "R2"
  Global_Vz/1 -> Wheel/10  "Global_Vz"
  Demux/1018 -> Global_Vz/1  "L1"
  Demux/1019 -> Global_Vz/2  "L2"
  Demux/1020 -> Global_Vz/3  "R1"
  Demux/1021 -> Global_Vz/4  "R2"
  Global_X/1 -> Wheel/11  "Global_X"
  Demux/1022 -> Global_X/1  "L1"
  Demux/1023 -> Global_X/2  "L2"
  Demux/1024 -> Global_X/3  "R1"
  Demux/1025 -> Global_X/4  "R2"
  Global_Y/1 -> Wheel/12  "Global_Y"
  Demux/1026 -> Global_Y/1  "L1"
  Demux/1027 -> Global_Y/2  "L2"
  Demux/1028 -> Global_Y/3  "R1"
  Demux/1029 -> Global_Y/4  "R2"
  Global_Z/1 -> Wheel/13  "Global_Z"
  Demux/1030 -> Global_Z/1  "L1"
  Demux/1031 -> Global_Z/2  "L2"
  Demux/1032 -> Global_Z/3  "R1"
  Demux/1033 -> Global_Z/4  "R2"
  Ground_Surface_Wheel_Center_Vx/1 -> Wheel/14  "Ground_Surface_Wheel_Center_Vx"
  Demux/1034 -> Ground_Surface_Wheel_Center_Vx/1  "L1"
  Demux/1035 -> Ground_Surface_Wheel_Center_Vx/2  "L2"
  Demux/1036 -> Ground_Surface_Wheel_Center_Vx/3  "R1"
  Demux/1037 -> Ground_Surface_Wheel_Center_Vx/4  "R2"
  Hub_Carrier_Omega_X/1 -> Wheel/15  "Hub_Carrier_Omega_X"
  Demux/1038 -> Hub_Carrier_Omega_X/1  "L1"
  Demux/1039 -> Hub_Carrier_Omega_X/2  "L2"
  Demux/1040 -> Hub_Carrier_Omega_X/3  "R1"
  Demux/1041 -> Hub_Carrier_Omega_X/4  "R2"
  Hub_Carrier_Omega_Y/1 -> Wheel/16  "Hub_Carrier_Omega_Y"
  Demux/1042 -> Hub_Carrier_Omega_Y/1  "L1"
  Demux/1043 -> Hub_Carrier_Omega_Y/2  "L2"
  Demux/1044 -> Hub_Carrier_Omega_Y/3  "R1"
  Demux/1045 -> Hub_Carrier_Omega_Y/4  "R2"
  Hub_Carrier_Omega_Z/1 -> Wheel/17  "Hub_Carrier_Omega_Z"
  Demux/1046 -> Hub_Carrier_Omega_Z/1  "L1"
  Demux/1047 -> Hub_Carrier_Omega_Z/2  "L2"
  Demux/1048 -> Hub_Carrier_Omega_Z/3  "R1"
  Demux/1049 -> Hub_Carrier_Omega_Z/4  "R2"
  Hub_Carrier_Vx/1 -> Wheel/18  "Hub_Carrier_Vx"
  Demux/1050 -> Hub_Carrier_Vx/1  "L1"
  Demux/1051 -> Hub_Carrier_Vx/2  "L2"
  Demux/1052 -> Hub_Carrier_Vx/3  "R1"
  Demux/1053 -> Hub_Carrier_Vx/4  "R2"
  Hub_Carrier_Vy/1 -> Wheel/19  "Hub_Carrier_Vy"
  Demux/1054 -> Hub_Carrier_Vy/1  "L1"
  Demux/1055 -> Hub_Carrier_Vy/2  "L2"
  Demux/1056 -> Hub_Carrier_Vy/3  "R1"
  Demux/1057 -> Hub_Carrier_Vy/4  "R2"
  Hub_Carrier_Vz/1 -> Wheel/20  "Hub_Carrier_Vz"
  Demux/1058 -> Hub_Carrier_Vz/1  "L1"
  Demux/1059 -> Hub_Carrier_Vz/2  "L2"
  Demux/1060 -> Hub_Carrier_Vz/3  "R1"
  Demux/1061 -> Hub_Carrier_Vz/4  "R2"
  hub_center_accx/1 -> Wheel/21  "hub_center_accx"
  Demux/1062 -> hub_center_accx/1  "front_left"
  Demux/1063 -> hub_center_accx/2  "front_right"
  Demux/1064 -> hub_center_accx/3  "rear_left"
  Demux/1065 -> hub_center_accx/4  "rear_right"
  hub_center_accy/1 -> Wheel/22  "hub_center_accy"
  Demux/1066 -> hub_center_accy/1  "front_left"
  Demux/1067 -> hub_center_accy/2  "front_right"
  Demux/1068 -> hub_center_accy/3  "rear_left"
  Demux/1069 -> hub_center_accy/4  "rear_right"
  hub_center_accz/1 -> Wheel/23  "hub_center_accz"
  Demux/1070 -> hub_center_accz/1  "front_left"
  Demux/1071 -> hub_center_accz/2  "front_right"
  Demux/1072 -> hub_center_accz/3  "rear_left"
  Demux/1073 -> hub_center_accz/4  "rear_right"
  Inclination/1 -> Wheel/24  "Inclination"
  Demux/1074 -> Inclination/1  "L1"
  Demux/1075 -> Inclination/2  "L2"
  Demux/1076 -> Inclination/3  "R1"
  Demux/1077 -> Inclination/4  "R2"
  Kingpin_Moment1/1 -> Wheel/25  "Kingpin_Moment"
  Demux/1078 -> Kingpin_Moment1/1  "L1"
  Demux/1079 -> Kingpin_Moment1/2  "R1"
  Omega/1 -> Wheel/26  "Omega"
  Demux/1080 -> Omega/1  "L1"
  Demux/1081 -> Omega/2  "L2"
  Demux/1082 -> Omega/3  "R1"
  Demux/1083 -> Omega/4  "R2"
  Phi/1 -> Wheel/27  "Phi"
  Demux/1084 -> Phi/1  "L1"
  Demux/1085 -> Phi/2  "L2"
  Demux/1086 -> Phi/3  "R1"
  Demux/1087 -> Phi/4  "R2"
  Pitch/1 -> Wheel/28  "Pitch"
  Demux/1088 -> Pitch/1  "L1"
  Demux/1089 -> Pitch/2  "L2"
  Demux/1090 -> Pitch/3  "R1"
  Demux/1091 -> Pitch/4  "R2"
  Psi/1 -> Wheel/29  "Psi"
  Demux/1092 -> Psi/1  "L1"
  Demux/1093 -> Psi/2  "L2"
  Demux/1094 -> Psi/3  "R1"
  Demux/1095 -> Psi/4  "R2"
  Rotation/1 -> Wheel/30  "Rotation"
  Demux/1096 -> Rotation/1  "L1"
  Demux/1097 -> Rotation/2  "L2"
  Demux/1098 -> Rotation/3  "R1"
  Demux/1099 -> Rotation/4  "R2"
  Side_View_Angle/1 -> Wheel/31  "Side_View_Angle"
  Demux/1100 -> Side_View_Angle/1  "L1"
  Demux/1101 -> Side_View_Angle/2  "L2"
  Demux/1102 -> Side_View_Angle/3  "R1"
  Demux/1103 -> Side_View_Angle/4  "R2"
  Spindle_Steer/1 -> Wheel/32  "Spindle_Steer"
  Demux/1104 -> Spindle_Steer/1  "L1"
  Demux/1105 -> Spindle_Steer/2  "L2"
  Demux/1106 -> Spindle_Steer/3  "R1"
  Demux/1107 -> Spindle_Steer/4  "R2"
  Theta/1 -> Wheel/33  "Theta"
  Demux/1108 -> Theta/1  "L1"
  Demux/1109 -> Theta/2  "L2"
  Demux/1110 -> Theta/3  "R1"
  Demux/1111 -> Theta/4  "R2"
  wheel_center_dispx/1 -> Wheel/34  "wheel_center_dispx"
  Demux/1112 -> wheel_center_dispx/1  "front_left"
  Demux/1113 -> wheel_center_dispx/2  "front_right"
  Demux/1114 -> wheel_center_dispx/3  "rear_left"
  Demux/1115 -> wheel_center_dispx/4  "rear_right"
  wheel_center_dispy/1 -> Wheel/35  "wheel_center_dispy"
  Demux/1116 -> wheel_center_dispy/1  "front_left"
  Demux/1117 -> wheel_center_dispy/2  "front_right"
  Demux/1118 -> wheel_center_dispy/3  "rear_left"
  Demux/1119 -> wheel_center_dispy/4  "rear_right"
  wheel_center_dispz/1 -> Wheel/36  "wheel_center_dispz"
  Demux/1120 -> wheel_center_dispz/1  "front_left"
  Demux/1121 -> wheel_center_dispz/2  "front_right"
  Demux/1122 -> wheel_center_dispz/3  "rear_left"
  Demux/1123 -> wheel_center_dispz/4  "rear_right"
  Yaw/1 -> Wheel/37  "Yaw"
  Demux/1124 -> Yaw/1  "L1"
  Demux/1125 -> Yaw/2  "L2"
  Demux/1126 -> Yaw/3  "R1"
  Demux/1127 -> Yaw/4  "R2"
  wheel_angles/1 -> OutputBus/76  "wheel_angles"
  Demux/1128 -> wheel_angles/1  "camber_L1"
  Demux/1129 -> wheel_angles/2  "camber_L2"
  Demux/1130 -> wheel_angles/3  "camber_R1"
  Demux/1131 -> wheel_angles/4  "camber_R2"
  Demux/1132 -> wheel_angles/5  "camber_wrt_road_L1"
  Demux/1133 -> wheel_angles/6  "camber_wrt_road_L2"
  Demux/1134 -> wheel_angles/7  "camber_wrt_road_R1"
  Demux/1135 -> wheel_angles/8  "camber_wrt_road_R2"
  Demux/1136 -> wheel_angles/9  "caster_L1"
  Demux/1137 -> wheel_angles/10  "caster_L2"
  Demux/1138 -> wheel_angles/11  "caster_R1"
  Demux/1139 -> wheel_angles/12  "caster_R2"
  Demux/1140 -> wheel_angles/13  "caster_wrt_road_L1"
  Demux/1141 -> wheel_angles/14  "caster_wrt_road_L2"
  Demux/1142 -> wheel_angles/15  "caster_wrt_road_R1"
  Demux/1143 -> wheel_angles/16  "caster_wrt_road_R2"
  Demux/1144 -> wheel_angles/17  "toe_L1"
  Demux/1145 -> wheel_angles/18  "toe_L2"
  Demux/1146 -> wheel_angles/19  "toe_R1"
  Demux/1147 -> wheel_angles/20  "toe_R2"
  Demux/1148 -> wheel_angles/21  "toe_wrt_road_L1"
  Demux/1149 -> wheel_angles/22  "toe_wrt_road_L2"
  Demux/1150 -> wheel_angles/23  "toe_wrt_road_R1"
  Demux/1151 -> wheel_angles/24  "toe_wrt_road_R2"
  whl_front_wheel_XFORM/1 -> OutputBus/77  "whl_front_wheel_XFORM"
  Demux/1152 -> whl_front_wheel_XFORM/1  "FX"
  Demux/1153 -> whl_front_wheel_XFORM/2  "FY"
  Demux/1154 -> whl_front_wheel_XFORM/3  "FZ"
  Demux/1155 -> whl_front_wheel_XFORM/4  "Phi"
  Demux/1156 -> whl_front_wheel_XFORM/5  "Psi"
  Demux/1157 -> whl_front_wheel_XFORM/6  "Theta"
  Demux/1158 -> whl_front_wheel_XFORM/7  "X"
  Demux/1159 -> whl_front_wheel_XFORM/8  "Y"
  Demux/1160 -> whl_front_wheel_XFORM/9  "Z"
  whl_rear_wheel_XFORM/1 -> OutputBus/78  "whl_rear_wheel_XFORM"
  Demux/1161 -> whl_rear_wheel_XFORM/1  "FX"
  Demux/1162 -> whl_rear_wheel_XFORM/2  "FY"
  Demux/1163 -> whl_rear_wheel_XFORM/3  "FZ"
  Demux/1164 -> whl_rear_wheel_XFORM/4  "Phi"
  Demux/1165 -> whl_rear_wheel_XFORM/5  "Psi"
  Demux/1166 -> whl_rear_wheel_XFORM/6  "Theta"
  Demux/1167 -> whl_rear_wheel_XFORM/7  "X"
  Demux/1168 -> whl_rear_wheel_XFORM/8  "Y"
  Demux/1169 -> whl_rear_wheel_XFORM/9  "Z"
  whl_twin_rear_wheel_XFORM/1 -> OutputBus/79  "whl_twin_rear_wheel_XFORM"
  Demux/1170 -> whl_twin_rear_wheel_XFORM/1  "FX"
  Demux/1171 -> whl_twin_rear_wheel_XFORM/2  "FY"
  Demux/1172 -> whl_twin_rear_wheel_XFORM/3  "FZ"
  Demux/1173 -> whl_twin_rear_wheel_XFORM/4  "Phi"
  Demux/1174 -> whl_twin_rear_wheel_XFORM/5  "Psi"
  Demux/1175 -> whl_twin_rear_wheel_XFORM/6  "Theta"
  Demux/1176 -> whl_twin_rear_wheel_XFORM/7  "X"
  Demux/1177 -> whl_twin_rear_wheel_XFORM/8  "Y"
  Demux/1178 -> whl_twin_rear_wheel_XFORM/9  "Z"
  whr_front_wheel_XFORM/1 -> OutputBus/80  "whr_front_wheel_XFORM"
  Demux/1179 -> whr_front_wheel_XFORM/1  "FX"
  Demux/1180 -> whr_front_wheel_XFORM/2  "FY"
  Demux/1181 -> whr_front_wheel_XFORM/3  "FZ"
  Demux/1182 -> whr_front_wheel_XFORM/4  "Phi"
  Demux/1183 -> whr_front_wheel_XFORM/5  "Psi"
  Demux/1184 -> whr_front_wheel_XFORM/6  "Theta"
  Demux/1185 -> whr_front_wheel_XFORM/7  "X"
  Demux/1186 -> whr_front_wheel_XFORM/8  "Y"
  Demux/1187 -> whr_front_wheel_XFORM/9  "Z"
  whr_rear_wheel_XFORM/1 -> OutputBus/81  "whr_rear_wheel_XFORM"
  Demux/1188 -> whr_rear_wheel_XFORM/1  "FX"
  Demux/1189 -> whr_rear_wheel_XFORM/2  "FY"
  Demux/1190 -> whr_rear_wheel_XFORM/3  "FZ"
  Demux/1191 -> whr_rear_wheel_XFORM/4  "Phi"
  Demux/1192 -> whr_rear_wheel_XFORM/5  "Psi"
  Demux/1193 -> whr_rear_wheel_XFORM/6  "Theta"
  Demux/1194 -> whr_rear_wheel_XFORM/7  "X"
  Demux/1195 -> whr_rear_wheel_XFORM/8  "Y"
  Demux/1196 -> whr_rear_wheel_XFORM/9  "Z"
  whr_twin_rear_wheel_XFORM/1 -> OutputBus/82  "whr_twin_rear_wheel_XFORM"
  Demux/1197 -> whr_twin_rear_wheel_XFORM/1  "FX"
  Demux/1198 -> whr_twin_rear_wheel_XFORM/2  "FY"
  Demux/1199 -> whr_twin_rear_wheel_XFORM/3  "FZ"
  Demux/1200 -> whr_twin_rear_wheel_XFORM/4  "Phi"
  Demux/1201 -> whr_twin_rear_wheel_XFORM/5  "Psi"
  Demux/1202 -> whr_twin_rear_wheel_XFORM/6  "Theta"
  Demux/1203 -> whr_twin_rear_wheel_XFORM/7  "X"
  Demux/1204 -> whr_twin_rear_wheel_XFORM/8  "Y"
  Demux/1205 -> whr_twin_rear_wheel_XFORM/9  "Z"
  Tire_front_left/1 -> OutputBus/83  "Tire_front_left"
  Demux/1206 -> Tire_front_left/1  "longitudinal_slip_actual"
  Demux/1207 -> Tire_front_left/2  "lateral_slip_actual"
  Demux/1208 -> Tire_front_left/3  "longitudinal_slip_kinematic_unbounded"
  Demux/1209 -> Tire_front_left/4  "lateral_slip_kinematic_unbounded"
  Demux/1210 -> Tire_front_left/5  "longitudinal_slip_transient_unbounded"
  Demux/1211 -> Tire_front_left/6  "lateral_slip_transient_unbounded"
  Tire_front_right/1 -> OutputBus/84  "Tire_front_right"
  Demux/1212 -> Tire_front_right/1  "longitudinal_slip_actual"
  Demux/1213 -> Tire_front_right/2  "lateral_slip_actual"
  Demux/1214 -> Tire_front_right/3  "longitudinal_slip_kinematic_unbounded"
  Demux/1215 -> Tire_front_right/4  "lateral_slip_kinematic_unbounded"
  Demux/1216 -> Tire_front_right/5  "longitudinal_slip_transient_unbounded"
  Demux/1217 -> Tire_front_right/6  "lateral_slip_transient_unbounded"
  Tire_rear_left/1 -> OutputBus/85  "Tire_rear_left"
  Demux/1218 -> Tire_rear_left/1  "longitudinal_slip_actual"
  Demux/1219 -> Tire_rear_left/2  "lateral_slip_actual"
  Demux/1220 -> Tire_rear_left/3  "longitudinal_slip_kinematic_unbounded"
  Demux/1221 -> Tire_rear_left/4  "lateral_slip_kinematic_unbounded"
  Demux/1222 -> Tire_rear_left/5  "longitudinal_slip_transient_unbounded"
  Demux/1223 -> Tire_rear_left/6  "lateral_slip_transient_unbounded"
  Tire_rear_right/1 -> OutputBus/86  "Tire_rear_right"
  Demux/1224 -> Tire_rear_right/1  "longitudinal_slip_actual"
  Demux/1225 -> Tire_rear_right/2  "lateral_slip_actual"
  Demux/1226 -> Tire_rear_right/3  "longitudinal_slip_kinematic_unbounded"
  Demux/1227 -> Tire_rear_right/4  "lateral_slip_kinematic_unbounded"
  Demux/1228 -> Tire_rear_right/5  "longitudinal_slip_transient_unbounded"
  Demux/1229 -> Tire_rear_right/6  "lateral_slip_transient_unbounded"
  Steering_Column/1 -> OutputBus/87  "Steering_Column"
  Demux/1230 -> Steering_Column/1  "steering_assist_force"
  Demux/1231 -> Steering_Column/2  "steering_assist_torque"
  Demux/1234 -> Steering_Column/3  "lower_column_rotation"
  Demux/1235 -> Steering_Column/4  "lower_column_rotational_velocity"
  Demux/1236 -> Steering_Column/5  "friction_torque"
  Demux/1237 -> Steering_Column/6  "upper_cardan_shaft_ratio"
  Demux/1238 -> Steering_Column/7  "middle_cardan_shaft_ratio"
  Demux/1239 -> Steering_Column/8  "lower_cardan_shaft_ratio"
  Demux/1240 -> Steering_Column/9  "overall_cardan_shaft_ratio"
  Demux/1241 -> Steering_Column/10  "inertial_torque"
  Demux/1242 -> Steering_Column/11  "steering_wheel_torque"
  Demux/1243 -> Steering_Column/12  "steering_wheel_torque_without_upper_inertia"
  Demux/1244 -> Steering_Column/13  "lower_column_deformation"
  Demux/1245 -> Steering_Column/14  "lower_column_deformation_velocity"
  Demux/1246 -> Steering_Column/15  "upper_column_deformation"
  Demux/1247 -> Steering_Column/16  "upper_column_deformation_velocity"
  Demux/1248 -> Steering_Column/17  "lower_column_stiffness_torque"
  Demux/1249 -> Steering_Column/18  "lower_column_damping_torque"
  Demux/1250 -> Steering_Column/19  "upper_column_stiffness_torque"
  Demux/1251 -> Steering_Column/20  "upper_column_damping_torque"
  Demux/1254 -> Steering_Column/21  "total_torque_upper_column"
  Demux/1255 -> Steering_Column/22  "total_torque_lower_column"
  Demux/1265 -> Steering_Column/23  "hardy_disc_deformation"
  Demux/1270 -> Steering_Column/24  "upper_column_angle"
  Demux/1271 -> Steering_Column/25  "upper_column_velocity"
  Demux/1272 -> Steering_Column/26  "lower_cardan_joint_output_rotation"
  Demux/1273 -> Steering_Column/27  "lower_cardan_joint_output_velocity"
  Demux/1274 -> Steering_Column/28  "middle_cardan_joint_output_rotation"
  Demux/1275 -> Steering_Column/29  "middle_cardan_joint_output_velocity"
  Demux/1276 -> Steering_Column/30  "upper_cardan_joint_output_rotation"
  Demux/1277 -> Steering_Column/31  "upper_cardan_joint_output_velocity"
  Demux/1282 -> Steering_Column/32  "simulator_steering_wheel_torque"
  Steering_Torsion_Bar/1 -> OutputBus/88  "Steering_Torsion_Bar"
  Demux/1232 -> Steering_Torsion_Bar/1  "torsion_bar_twist_angle"
  Demux/1252 -> Steering_Torsion_Bar/2  "friction_torque"
  Demux/1253 -> Steering_Torsion_Bar/3  "torsion_bar_twist_angle_saturated"
  Demux/1278 -> Steering_Torsion_Bar/4  "torsion_bar_deformation_velocity"
  Demux/1279 -> Steering_Torsion_Bar/5  "torsion_bar_load"
  Steering_Rack_Pinion/1 -> OutputBus/89  "Steering_Rack_Pinion"
  Demux/1256 -> Steering_Rack_Pinion/1  "rack_displacement_saturated"
  Demux/1257 -> Steering_Rack_Pinion/2  "pinion_rotation"
  Demux/1258 -> Steering_Rack_Pinion/3  "pinion_rotational_velocity"
  Demux/1259 -> Steering_Rack_Pinion/4  "rack_force_from_lower_column"
  Demux/1260 -> Steering_Rack_Pinion/5  "rack_friction_force"
  Demux/1261 -> Steering_Rack_Pinion/6  "rack_acceleration"
  Demux/1267 -> Steering_Rack_Pinion/7  "total_rack_mass"
  Demux/1268 -> Steering_Rack_Pinion/8  "rack_total_force"
  Demux/1269 -> Steering_Rack_Pinion/9  "rack_velocity"
  Demux/1280 -> Steering_Rack_Pinion/10  "rack_force"
  Demux/1283 -> Steering_Rack_Pinion/11  "rack_displacement"
  Motor/1 -> OutputBus/90  "Motor"
  Demux/1262 -> Motor/1  "motor_angle"
  Demux/1263 -> Motor/2  "motor_velocity"
  Demux/1264 -> Motor/3  "motor_torque"
  Demux/1266 -> Motor/4  "motor_current"
  Demux/1286 -> Motor/5  "motor_friction"
  path_sensor/1 -> OutputBus/91  "path_sensor"
  Demux/1293 -> path_sensor/1  "total_lap_time"
  Demux/1294 -> path_sensor/2  "total_lap_count"
  Demux/1295 -> path_sensor/3  "last_sector_time"
  Demux/1296 -> path_sensor/4  "progressive_time"
  Demux/1297 -> path_sensor/5  "path_s"
  Demux/1298 -> path_sensor/6  "path_distance"
  Animator_Widget/1 -> OutputBus/92  "Animator_Widget"
  Demux/1299 -> Animator_Widget/1  "longitudinal_speed"
  Demux/1300 -> Animator_Widget/2  "engine_rpm"
  ges_hub_XFORMFL/1 -> OutputBus/93  "ges_hub_XFORMFL"
  Demux/1302 -> ges_hub_XFORMFL/1  "X"
  Demux/1303 -> ges_hub_XFORMFL/2  "Y"
  Demux/1304 -> ges_hub_XFORMFL/3  "Z"
  Demux/1305 -> ges_hub_XFORMFL/4  "Psi"
  Demux/1306 -> ges_hub_XFORMFL/5  "Theta"
  Demux/1307 -> ges_hub_XFORMFL/6  "Phi"
  hub2cp_XFORMFL/1 -> OutputBus/94  "hub2cp_XFORMFL"
  Demux/1308 -> hub2cp_XFORMFL/1  "X"
  Demux/1309 -> hub2cp_XFORMFL/2  "Y"
  Demux/1310 -> hub2cp_XFORMFL/3  "Z"
  cp_force_longitudinalFL/1 -> OutputBus/95  "cp_force_longitudinalFL"
  Demux/1311 -> cp_force_longitudinalFL/1  "X"
  Demux/1312 -> cp_force_longitudinalFL/2  "Y"
  Demux/1313 -> cp_force_longitudinalFL/3  "Z"
  cp_force_lateralFL/1 -> OutputBus/96  "cp_force_lateralFL"
  Demux/1314 -> cp_force_lateralFL/1  "X"
  Demux/1315 -> cp_force_lateralFL/2  "Y"
  Demux/1316 -> cp_force_lateralFL/3  "Z"
  cp_force_normalFL/1 -> OutputBus/97  "cp_force_normalFL"
  Demux/1317 -> cp_force_normalFL/1  "X"
  Demux/1318 -> cp_force_normalFL/2  "Y"
  Demux/1319 -> cp_force_normalFL/3  "Z"
  ges_hub_XFORMFR/1 -> OutputBus/98  "ges_hub_XFORMFR"
  Demux/1320 -> ges_hub_XFORMFR/1  "X"
  Demux/1321 -> ges_hub_XFORMFR/2  "Y"
  Demux/1322 -> ges_hub_XFORMFR/3  "Z"
  Demux/1323 -> ges_hub_XFORMFR/4  "Psi"
  Demux/1324 -> ges_hub_XFORMFR/5  "Theta"
  Demux/1325 -> ges_hub_XFORMFR/6  "Phi"
  hub2cp_XFORMFR/1 -> OutputBus/99  "hub2cp_XFORMFR"
  Demux/1326 -> hub2cp_XFORMFR/1  "X"
  Demux/1327 -> hub2cp_XFORMFR/2  "Y"
  Demux/1328 -> hub2cp_XFORMFR/3  "Z"
  cp_force_longitudinalFR/1 -> OutputBus/100  "cp_force_longitudinalFR"
  Demux/1329 -> cp_force_longitudinalFR/1  "X"
  Demux/1330 -> cp_force_longitudinalFR/2  "Y"
  Demux/1331 -> cp_force_longitudinalFR/3  "Z"
  cp_force_lateralFR/1 -> OutputBus/101  "cp_force_lateralFR"
  Demux/1332 -> cp_force_lateralFR/1  "X"
  Demux/1333 -> cp_force_lateralFR/2  "Y"
  Demux/1334 -> cp_force_lateralFR/3  "Z"
  cp_force_normalFR/1 -> OutputBus/102  "cp_force_normalFR"
  Demux/1335 -> cp_force_normalFR/1  "X"
  Demux/1336 -> cp_force_normalFR/2  "Y"
  Demux/1337 -> cp_force_normalFR/3  "Z"
  ges_hub_XFORMRL/1 -> OutputBus/103  "ges_hub_XFORMRL"
  Demux/1338 -> ges_hub_XFORMRL/1  "X"
  Demux/1339 -> ges_hub_XFORMRL/2  "Y"
  Demux/1340 -> ges_hub_XFORMRL/3  "Z"
  Demux/1341 -> ges_hub_XFORMRL/4  "Psi"
  Demux/1342 -> ges_hub_XFORMRL/5  "Theta"
  Demux/1343 -> ges_hub_XFORMRL/6  "Phi"
  hub2cp_XFORMRL/1 -> OutputBus/104  "hub2cp_XFORMRL"
  Demux/1344 -> hub2cp_XFORMRL/1  "X"
  Demux/1345 -> hub2cp_XFORMRL/2  "Y"
  Demux/1346 -> hub2cp_XFORMRL/3  "Z"
  cp_force_longitudinalRL/1 -> OutputBus/105  "cp_force_longitudinalRL"
  Demux/1347 -> cp_force_longitudinalRL/1  "X"
  Demux/1348 -> cp_force_longitudinalRL/2  "Y"
  Demux/1349 -> cp_force_longitudinalRL/3  "Z"
  cp_force_lateralRL/1 -> OutputBus/106  "cp_force_lateralRL"
  Demux/1350 -> cp_force_lateralRL/1  "X"
  Demux/1351 -> cp_force_lateralRL/2  "Y"
  Demux/1352 -> cp_force_lateralRL/3  "Z"
  cp_force_normalRL/1 -> OutputBus/107  "cp_force_normalRL"
  Demux/1353 -> cp_force_normalRL/1  "X"
  Demux/1354 -> cp_force_normalRL/2  "Y"
  Demux/1355 -> cp_force_normalRL/3  "Z"
  ges_hub_XFORMRR/1 -> OutputBus/108  "ges_hub_XFORMRR"
  Demux/1356 -> ges_hub_XFORMRR/1  "X"
  Demux/1357 -> ges_hub_XFORMRR/2  "Y"
  Demux/1358 -> ges_hub_XFORMRR/3  "Z"
  Demux/1359 -> ges_hub_XFORMRR/4  "Psi"
  Demux/1360 -> ges_hub_XFORMRR/5  "Theta"
  Demux/1361 -> ges_hub_XFORMRR/6  "Phi"
  hub2cp_XFORMRR/1 -> OutputBus/109  "hub2cp_XFORMRR"
  Demux/1362 -> hub2cp_XFORMRR/1  "X"
  Demux/1363 -> hub2cp_XFORMRR/2  "Y"
  Demux/1364 -> hub2cp_XFORMRR/3  "Z"
  cp_force_longitudinalRR/1 -> OutputBus/110  "cp_force_longitudinalRR"
  Demux/1365 -> cp_force_longitudinalRR/1  "X"
  Demux/1366 -> cp_force_longitudinalRR/2  "Y"
  Demux/1367 -> cp_force_longitudinalRR/3  "Z"
  cp_force_lateralRR/1 -> OutputBus/111  "cp_force_lateralRR"
  Demux/1368 -> cp_force_lateralRR/1  "X"
  Demux/1369 -> cp_force_lateralRR/2  "Y"
  Demux/1370 -> cp_force_lateralRR/3  "Z"
  cp_force_normalRR/1 -> OutputBus/112  "cp_force_normalRR"
  Demux/1371 -> cp_force_normalRR/1  "X"
  Demux/1372 -> cp_force_normalRR/2  "Y"
  Demux/1373 -> cp_force_normalRR/3  "Z"
  Road_Material/1 -> OutputBus/113  "Road_Material"
  Demux/1374 -> Road_Material/1  "front_left_tire"
  Demux/1375 -> Road_Material/2  "front_right_tire"
  Demux/1376 -> Road_Material/3  "rear_left_tire"
  Demux/1377 -> Road_Material/4  "rear_right_tire"
